simulink library "ammclib_bam_S32K3xx"  (R2016a)
settings: Solver=VariableStepAuto  SolverMode=SingleTasking  StartTime=0.0  StopTime=10.0  RelTol=1e-3
undefined symbols (not defined in the file or in its folder): a1, a2, ADCMaxError, autoCalcEn, b0, b1, b2, cfg, dgain, escale, f16A1, f16A2, f16ADCMaxError, f16B0, f16B1, f16B2, f16C1, f16CC1sc, f16CC1sc_D, f16CC1sc_Q, f16CC2sc, f16CC2sc_D, f16CC2sc_Q, f16DerivGain, f16EGain, f16FiltCoef, f16HystOff, f16HystOn, f16IGain, f16IntegGain, f16IntegGain_D, f16IntegGain_Q, f16IntegGainQ, f16Kd, f16KLs, f16Kq, f16KRs, f16Limit, f16LowerLimit, f16LowerLimit_D, f16LowerLimit_Q, f16LowerLimitQ, f16ModIndex, f16OutValOff, f16OutValOn, f16PropGain, f16PropGain_D, f16PropGain_Q, f16PropGainQ, f16RampDown, f16RampUp, f16UGain, f16UpperLimit, f16UpperLimit_D, f16UpperLimit_Q, f16UpperLimitQ, f16WIGain, f32A1, f32A2, f32ADCMaxError ... (+180)
(part 22 of 50)

== system ammclib_bam_S32K3xx/AMCLIB/FLT ==
  AMCLIB_BemfObsrvDQ_FLT : Subsystem  StartFcn=|  TreatAsAtomicUnit=on  mask(AMCLIB_BemfObsrvDQ_FLT){showStates=Hide (faster execution), resetStatesEnable=Pre-set according to the first set of inputs after reset, SampleTime=-1, intmethod=Trapezoidal, if0=350, iksi=1, Ld=3e-4, Lq=3e-4, Rs=0.33, mechspeed=3000, polepairs=1, autoCalcEn=on, fltIGain=0, fltUGain=0, fltWIGain=0, fltEGain=0, fltCC1sc_D=0, fltCC2sc_D=0, fltUpperLimit_D=0, fltLowerLimit_D=0, fltCC1sc_Q=0, fltCC2sc_Q=0, fltUpperLimit_Q=0, fltLowerLimit_Q=0, SampleTime_1=NaN}
      | ts=get_param(gcb,'CompiledSampleTime');
      | if iscell(ts)
      |   ts=ts{1};
      |   if iscell(ts)
      |     ts=ts{1};
      |   end
      | end
      | ts=ts(1);
      | set_param(gcb,'SampleTime_1',num2str(ts));
      | p=Simulink.Mask.get(gcb);
      | hintText=p.getDialogControl('timeHint');
      | SampleTime=Simulink.data.evalinGlobal(bdroot,get_param(gcb,'SampleTime'));
      | p=Simulink.Mask.get(gcb);
      | autoCalcEn=get_param(gcb,'autoCalcEn');
      | if strcmp(autoCalcEn,'on')
      |   if SampleTime==-1
      |     hintText.Prompt='Caution: Implementation parameters depend on inherited sample time. Make sure that the sample time of the block''s inputs corresponds to the sampling period in the target application.';
      |   else
      |     hintText.Prompt='Caution: Implementation parameters depend on the sample time. Make sure that the simulation time step corresponds to the sampling period in the target application.';
      |   end
      |   SampleTime=ts;
      |   fltIGain_bkup=get_param(gcb,'fltIGain');
      |   fltUGain_bkup=get_param(gcb,'fltUGain');
      |   fltWIGain_bkup=get_param(gcb,'fltWIGain');
      |   fltEGain_bkup=get_param(gcb,'fltEGain');
      |   fltCC1sc_D_bkup=get_param(gcb,'fltCC1sc_D');
      |   fltCC2sc_D_bkup=get_param(gcb,'fltCC2sc_D');
      |   fltUpperLimit_D_bkup=get_param(gcb,'fltUpperLimit_D');
      |   fltLowerLimit_D_bkup=get_param(gcb,'fltLowerLimit_D');
      |   fltCC1sc_Q_bkup=get_param(gcb,'fltCC1sc_Q');
      |   fltCC2sc_Q_bkup=get_param(gcb,'fltCC2sc_Q');
      |   fltUpperLimit_Q_bkup=get_param(gcb,'fltUpperLimit_Q');
      |   fltLowerLimit_Q_bkup=get_param(gcb,'fltLowerLimit_Q');
      |   intmethod=get_param(gcb,'intmethod');
      |   if0=Simulink.data.evalinGlobal(bdroot,get_param(gcb,'if0'));
      |   iksi=Simulink.data.evalinGlobal(bdroot,get_param(gcb,'iksi'));
      |   Ld=Simulink.data.evalinGlobal(bdroot,get_param(gcb,'Ld'));
      |   Lq=Simulink.data.evalinGlobal(bdroot,get_param(gcb,'Lq'));
      |   Rs=Simulink.data.evalinGlobal(bdroot,get_param(gcb,'Rs'));
      |   mechspeed=Simulink.data.evalinGlobal(bdroot,get_param(gcb,'mechspeed'));
      |   polepairs=Simulink.data.evalinGlobal(bdroot,get_param(gcb,'polepairs'));
      |   if (if0<=0)
      |     warning('Natural frequency f0 must be positive.');
      |   end
      |   if (iksi<=0)
      |     warning('Current loop attenuation must be positive.');
      |   end
      |   if (iksi>1)
      |     warning('Current loop attenuation must not exceed 1.');
      |   end
      |   if (Ld<=0)
      |     warning('Inductance Ld must be positive.');
      |   end
      |   if (Lq<=0)
      |     warning('Inductance Lq must be positive.');
      |   end
      |   if (Rs<0)
      |     warning('Resistance Rs must be non-negative.');
      |   end
      |   if (mechspeed<=0)
      |     warning('Max. speed must be positive.');
      |   end
      |   if (polepairs<1)
      |     warning('Number of pole pairs must be a natural number (1, 2, 3, ...).');
      |   end
      |   if (round(polepairs)~=polepairs)
      |     warning('Number of pole pairs must be a natural number (1, 2, 3, ...).');
      |   end
      |   w0=6.283185307179586*if0;
      |   pgain=2.0*iksi*w0*Ld-Rs;
      |   igain=w0*w0*Ld;
      |   if strcmp(intmethod,'Forward Rectangular')
      |     cc1=pgain;
      |     cc2=-pgain+igain*SampleTime;
      |   else
      |     if strcmp(intmethod,'Backward Rectangular')
      |       cc1=pgain+igain*SampleTime;
      |       cc2=-pgain;
      |     else
      |       cc1=pgain+igain*SampleTime*0.5;
      |       cc2=-pgain+igain*SampleTime*0.5;
      |     end
      |   end
      |   fltCC1sc_D=cc1;
      |   fltCC2sc_D=cc2;
      |   fltCC1sc_Q=fltCC1sc_D;
      |   fltCC2sc_Q=fltCC2sc_D;
      |   fltLowerLimit_D=-1000000.0;
      |   fltUpperLimit_D=1000000.0;
      |   fltLowerLimit_Q=fltLowerLimit_D;
      |   fltUpperLimit_Q=fltUpperLimit_D;
      |   fltIGain=(2.0*Ld-SampleTime*Rs)/(2.0*Ld+SampleTime*Rs);
      |   fltUGain=SampleTime/(2.0*Ld+SampleTime*Rs);
      |   fltWIGain=SampleTime*Lq/(2.0*Ld+SampleTime*Rs);
      |   fltEGain=SampleTime/(2.0*Ld+SampleTime*Rs);
      |   if isnan(fltIGain)
      |     if ~strcmp(fltIGain_bkup,'0')
      |       set_param(gcb,'fltIGain','0');
      |     end
      |   else
      |     tmps=num2str(fltIGain);
      |     if ~strcmp(fltIGain_bkup,tmps)
      |       set_param(gcb,'fltIGain',tmps);
      |     end
      |   end
      |   if isnan(fltUGain)
      |     if ~strcmp(fltUGain_bkup,'0')
      |       set_param(gcb,'fltUGain','0');
      |     end
      |   else
      |     tmps=num2str(fltUGain);
      |     if ~strcmp(fltUGain_bkup,tmps)
      |       set_param(gcb,'fltUGain',tmps);
      |     end
      |   end
      |   if isnan(fltWIGain)
      |     if ~strcmp(fltWIGain_bkup,'0')
      |       set_param(gcb,'fltWIGain','0');
      |     end
      |   else
      |     tmps=num2str(fltWIGain);
      |     if ~strcmp(fltWIGain_bkup,tmps)
      |       set_param(gcb,'fltWIGain',tmps);
      |     end
      |   end
      |   if isnan(fltEGain)
      |     if ~strcmp(fltEGain_bkup,'0')
      |       set_param(gcb,'fltEGain','0');
      |     end
      |   else
      |     tmps=num2str(fltEGain);
      |     if ~strcmp(fltEGain_bkup,tmps)
      |       set_param(gcb,'fltEGain',tmps);
      |     end
      |   end
      |   if isnan(fltCC1sc_D)
      |     if ~strcmp(fltCC1sc_D_bkup,'0')
      |       set_param(gcb,'fltCC1sc_D','0');
      |     end
      |   else
      |     tmps=num2str(fltCC1sc_D);
      |     if ~strcmp(fltCC1sc_D_bkup,tmps)
      |       set_param(gcb,'fltCC1sc_D',tmps);
      |     end
      |   end
      |   if isnan(fltCC2sc_D)
      |     if ~strcmp(fltCC2sc_D_bkup,'0')
      |       set_param(gcb,'fltCC2sc_D','0');
      |     end
      |   else
      |     tmps=num2str(fltCC2sc_D);
      |     if ~strcmp(fltCC2sc_D_bkup,tmps)
      |       set_param(gcb,'fltCC2sc_D',tmps);
      |     end
      |   end
      |   if isnan(fltUpperLimit_D)
      |     if ~strcmp(fltUpperLimit_D_bkup,'0')
      |       set_param(gcb,'fltUpperLimit_D','0');
      |     end
      |   else
      |     tmps=num2str(fltUpperLimit_D);
      |     if ~strcmp(fltUpperLimit_D_bkup,tmps)
      |       set_param(gcb,'fltUpperLimit_D',tmps);
      |     end
      |   end
      |   if isnan(fltLowerLimit_D)
      |     if ~strcmp(fltLowerLimit_D_bkup,'0')
      |       set_param(gcb,'fltLowerLimit_D','0');
      |     end
      |   else
      |     tmps=num2str(fltLowerLimit_D);
      |     if ~strcmp(fltLowerLimit_D_bkup,tmps)
      |       set_param(gcb,'fltLowerLimit_D',tmps);
      |     end
      |   end
      |   if isnan(fltCC1sc_Q)
      |     if ~strcmp(fltCC1sc_Q_bkup,'0')
      |       set_param(gcb,'fltCC1sc_Q','0');
      |     end
      |   else
      |     tmps=num2str(fltCC1sc_Q);
      |     if ~strcmp(fltCC1sc_Q_bkup,tmps)
      |       set_param(gcb,'fltCC1sc_Q',tmps);
      |     end
      |   end
      |   if isnan(fltCC2sc_Q)
      |     if ~strcmp(fltCC2sc_Q_bkup,'0')
      |       set_param(gcb,'fltCC2sc_Q','0');
      |     end
      |   else
      |     tmps=num2str(fltCC2sc_Q);
      |     if ~strcmp(fltCC2sc_Q_bkup,tmps)
      |       set_param(gcb,'fltCC2sc_Q',tmps);
      |     end
      |   end
      |   if isnan(fltUpperLimit_Q)
      |     if ~strcmp(fltUpperLimit_Q_bkup,'0')
      |       set_param(gcb,'fltUpperLimit_Q','0');
      |     end
      |   else
      |     tmps=num2str(fltUpperLimit_Q);
      |     if ~strcmp(fltUpperLimit_Q_bkup,tmps)
      |       set_param(gcb,'fltUpperLimit_Q',tmps);
      |     end
      |   end
      |   if isnan(fltLowerLimit_Q)
      |     if ~strcmp(fltLowerLimit_Q_bkup,'0')
      |       set_param(gcb,'fltLowerLimit_Q','0');
      |     end
      |   else
      |     tmps=num2str(fltLowerLimit_Q);
      |     if ~strcmp(fltLowerLimit_Q_bkup,tmps)
      |       set_param(gcb,'fltLowerLimit_Q',tmps);
      |     end
      |   end
      | end
      mask prompts: showStates "Show internal states:"; resetStatesEnable "Internal state after reset:"; SampleTime "Sample time (-1 for inherited):"; intmethod "Integration method:"; if0 "Current loop natural frequency f0 [Hz]:"; iksi "Current loop attenuation ξ:"; Ld "D-axis stator inductance Ld [H]"; Lq "Q-axis stator inductance Lq [H]"; Rs "Winding resistance Rs [ohm]:"; mechspeed "Maximum mechanical speed of the motor [RPM]:"; polepairs "Number of pole pairs of the motor:"; autoCalcEn "Calculate implementation parameters from physical parameters"; fltIGain "fltIGain (RL circuit constant):"; fltUGain "fltUGain (Voltage cross-coupling constant):"; fltWIGain "fltWIGain (Angular velocity cross-coupling constant):"; fltEGain "fltEGain (Back-EMF cross-coupling constant):"; fltCC1sc_D "fltCC1sc_D (CC1 coefficient of the D-axis PI controller):"; fltCC2sc_D "fltCC2sc_D (CC2 coefficient of the D-axis PI controller):"; fltUpperLimit_D "fltUpperLimit_D (Upper Limit of the D-axis PI controller):"; fltLowerLimit_D "fltLowerLimit_D (Lower Limit of the D-axis PI controller):"; fltCC1sc_Q "fltCC1sc_Q (CC1 coefficient of the Q-axis PI controller):"; fltCC2sc_Q "fltCC2sc_Q (CC2 coefficient of the Q-axis PI controller):"; fltUpperLimit_Q "fltUpperLimit_Q (Upper Limit of the Q-axis PI controller):"; fltLowerLimit_Q "fltLowerLimit_Q (Lower Limit of the Q-axis PI controller):"; SampleTime_1 "Discrete sample time:"
      mask help: PMSM back-EMF observer DQ in single precision floating-point implementation. This block supports re-initialization of the internal state during simulation. If the block is reset, the observer will align with the motor's position and speed measured in the next time step. This allows seamless on-the-fly transition to the closed-loop control. Refer to the AMMCLIB User's Guide for further details.
      mask init:
      | ddName = get_param(bdroot,'DataDictionary');
      | if length(ddName)==0
      |   set_param(bdroot,'DataDictionary','ammclib_types.sldd');
      | else
      |   dd = Simulink.data.dictionary.open(ddName);
      |   data = getSection(dd,'Design Data');
      |   if ~exist(data,'SWLIBS_2Syst_F16')
      |     addDataSource(dd,'ammclib_types.sldd');
      |     saveChanges(dd);
      |   end
      | end
      | 
      | if showStates == 1
      |   % hidden state variables
      |   if strcmp(get_param([gcb '/fltIGain'], 'BlockType'), 'Inport')
      |     posblk = get_param(gcb, 'Position');
      | 
      |     pos = get_param([gcb, '/fltIGain'], 'Position');
      |     orient = get_param([gcb, '/fltIGain'], 'Orientation');
      |     delete_block([gcb, '/fltIGain']);
      |     add_block('built-in/Ground', [gcb, '/fltIGain'], 'Position', pos, 'Orientation', orient);
      | 
      |     pos = get_param([gcb, '/fltUGain'], 'Position');
      |     orient = get_param([gcb, '/fltUGain'], 'Orientation');
      |     delete_block([gcb, '/fltUGain']);
      |     add_block('built-in/Ground', [gcb, '/fltUGain'], 'Position', pos, 'Orientation', orient);
      | 
      |     pos = get_param([gcb, '/fltWIGain'], 'Position');
      |     orient = get_param([gcb, '/fltWIGain'], 'Orientation');
      |     delete_block([gcb, '/fltWIGain']);
      |     add_block('built-in/Ground', [gcb, '/fltWIGain'], 'Position', pos, 'Orientation', orient);
      | 
      |     pos = get_param([gcb, '/fltEGain'], 'Position');
      |     orient = get_param([gcb, '/fltEGain'], 'Orientation');
      |     delete_block([gcb, '/fltEGain']);
      |     add_block('built-in/Ground', [gcb, '/fltEGain'], 'Position', pos, 'Orientation', orient);
      | 
      |     pos = get_param([gcb, '/fltCC1sc_D'], 'Position');
      |     orient = get_param([gcb, '/fltCC1sc_D'], 'Orientation');
      |     delete_block([gcb, '/fltCC1sc_D']);
      |     add_block('built-in/Ground', [gcb, '/fltCC1sc_D'], 'Position', pos, 'Orientation', orient);
      | 
      |     pos = get_param([gcb, '/fltCC2sc_D'], 'Position');
      |     orient = get_param([gcb, '/fltCC2sc_D'], 'Orientation');
      |     delete_block([gcb, '/fltCC2sc_D']);
      |     add_block('built-in/Ground', [gcb, '/fltCC2sc_D'], 'Position', pos, 'Orientation', orient);
      | 
      |     pos = get_param([gcb, '/fltUpperLimit_D'], 'Position');
      |     orient = get_param([gcb, '/fltUpperLimit_D'], 'Orientation');
      |     delete_block([gcb, '/fltUpperLimit_D']);
      |     add_block('built-in/Ground', [gcb, '/fltUpperLimit_D'], 'Position', pos, 'Orientation', orient);
      | 
      |     pos = get_param([gcb, '/fltLowerLimit_D'], 'Position');
      |     orient = get_param([gcb, '/fltLowerLimit_D'], 'Orientation');
      |     delete_block([gcb, '/fltLowerLimit_D']);
      |     add_block('built-in/Ground', [gcb, '/fltLowerLimit_D'], 'Position', pos, 'Orientation', orient);
      | 
      |     pos = get_param([gcb, '/fltCC1sc_Q'], 'Position');
      |     orient = get_param([gcb, '/fltCC1sc_Q'], 'Orientation');
      |     delete_block([gcb, '/fltCC1sc_Q']);
      |     add_block('built-in/Ground', [gcb, '/fltCC1sc_Q'], 'Position', pos, 'Orientation', orient);
      | 
      |     pos = get_param([gcb, '/fltCC2sc_Q'], 'Position');
      |     orient = get_param([gcb, '/fltCC2sc_Q'], 'Orientation');
      |     delete_block([gcb, '/fltCC2sc_Q']);
      |     add_block('built-in/Ground', [gcb, '/fltCC2sc_Q'], 'Position', pos, 'Orientation', orient);
      | 
      |     pos = get_param([gcb, '/fltUpperLimit_Q'], 'Position');
      |     orient = get_param([gcb, '/fltUpperLimit_Q'], 'Orientation');
      |     delete_block([gcb, '/fltUpperLimit_Q']);
      |     add_block('built-in/Ground', [gcb, '/fltUpperLimit_Q'], 'Position', pos, 'Orientation', orient);
      | 
      |     pos = get_param([gcb, '/fltLowerLimit_Q'], 'Position');
      |     orient = get_param([gcb, '/fltLowerLimit_Q'], 'Orientation');
      |     delete_block([gcb, '/fltLowerLimit_Q']);
      |     add_block('built-in/Ground', [gcb, '/fltLowerLimit_Q'], 'Position', pos, 'Orientation', orient);
      | 
      |     pos = get_param([gcb, '/fltAcc_D'], 'Position');
      |     orient = get_param([gcb, '/fltAcc_D'], 'Orientation');
      |     delete_block([gcb, '/fltAcc_D']);
      |     add_block('built-in/Ground', [gcb, '/fltAcc_D'], 'Position', pos, 'Orientation', orient);
      | 
      |     pos = get_param([gcb, '/fltInErrK1_D'], 'Position');
      |     orient = get_param([gcb, '/fltInErrK1_D'], 'Orientation');
      |     delete_block([gcb, '/fltInErrK1_D']);
      |     add_block('built-in/Ground', [gcb, '/fltInErrK1_D'], 'Position', pos, 'Orientation', orient);
      | 
      |     pos = get_param([gcb, '/fltAcc_Q'], 'Position');
      |     orient = get_param([gcb, '/fltAcc_Q'], 'Orientation');
      |     delete_block([gcb, '/fltAcc_Q']);
      |     add_block('built-in/Ground', [gcb, '/fltAcc_Q'], 'Position', pos, 'Orientation', orient);
      | 
      |     pos = get_param([gcb, '/fltInErrK1_Q'], 'Position');
      |     orient = get_param([gcb, '/fltInErrK1_Q'], 'Orientation');
      |     delete_block([gcb, '/fltInErrK1_Q']);
      |     add_block('built-in/Ground', [gcb, '/fltInErrK1_Q'], 'Position', pos, 'Orientation', orient);
      | 
      |     pos = get_param([gcb, '/fltIObsrvIn_1_D'], 'Position');
      |     orient = get_param([gcb, '/fltIObsrvIn_1_D'], 'Orientation');
      |     delete_block([gcb, '/fltIObsrvIn_1_D']);
      |     add_block('built-in/Ground', [gcb, '/fltIObsrvIn_1_D'], 'Position', pos, 'Orientation', orient);
      | 
      |     pos = get_param([gcb, '/fltIObsrvIn_1_Q'], 'Position');
      |     orient = get_param([gcb, '/fltIObsrvIn_1_Q'], 'Orientation');
      |     delete_block([gcb, '/fltIObsrvIn_1_Q']);
      |     add_block('built-in/Ground', [gcb, '/fltIObsrvIn_1_Q'], 'Position', pos, 'Orientation', orient);
      | 
      |     pos = get_param([gcb, '/fltIObsrv_D'], 'Position');
      |     orient = get_param([gcb, '/fltIObsrv_D'], 'Orientation');
      |     delete_block([gcb, '/fltIObsrv_D']);
      |     add_block('built-in/Ground', [gcb, '/fltIObsrv_D'], 'Position', pos, 'Orientation', orient);
      | 
      |     pos = get_param([gcb, '/fltIObsrv_Q'], 'Position');
      |     orient = get_param([gcb, '/fltIObsrv_Q'], 'Orientation');
      |     delete_block([gcb, '/fltIObsrv_Q']);
      |     add_block('built-in/Ground', [gcb, '/fltIObsrv_Q'], 'Position', pos, 'Orientation', orient);
      | 
      | 
      |     pmask=Simulink.Mask.get(gcb);
      |     pctrl=pmask.getParameter('SampleTime');
      |     pctrl.set('TypeOptions',{'pIAB/SampleTime','pUAB/SampleTime','fltVelocity/SampleTime','fltPhase/SampleTime'});
      | 
      |     pos = get_param([gcb '/fltEObsrv_D_Out'], 'Position');
      |     orient = get_param([gcb '/fltEObsrv_D_Out'], 'Orientation');
      |     delete_block([gcb '/fltEObsrv_D_Out']);
      |     add_block('built-in/Terminator', [gcb '/fltEObsrv_D_Out'], 'Position', pos, 'Orientation', orient);
      | 
      |     pos = get_param([gcb '/fltEObsrv_Q_Out'], 'Position');
      |     orient = get_param([gcb '/fltEObsrv_Q_Out'], 'Orientation');
      |     delete_block([gcb '/fltEObsrv_Q_Out']);
      |     add_block('built-in/Terminator', [gcb '/fltEObsrv_Q_Out'], 'Position', pos, 'Orientation', orient);
      | 
      |     pos = get_param([gcb '/fltAcc_D_Out'], 'Position');
      |     orient = get_param([gcb '/fltAcc_D_Out'], 'Orientation');
      |     delete_block([gcb '/fltAcc_D_Out']);
      |     add_block('built-in/Terminator', [gcb '/fltAcc_D_Out'], 'Position', pos, 'Orientation', orient);
      | 
      |     pos = get_param([gcb '/fltInErrK1_D_Out'], 'Position');
      |     orient = get_param([gcb '/fltInErrK1_D_Out'], 'Orientation');
      |     delete_block([gcb '/fltInErrK1_D_Out']);
      |     add_block('built-in/Terminator', [gcb '/fltInErrK1_D_Out'], 'Position', pos, 'Orientation', orient);
      | 
      |     pos = get_param([gcb '/fltAcc_Q_Out'], 'Position');
      |     orient = get_param([gcb '/fltAcc_Q_Out'], 'Orientation');
      |     delete_block([gcb '/fltAcc_Q_Out']);
      |     add_block('built-in/Terminator', [gcb '/fltAcc_Q_Out'], 'Position', pos, 'Orientation', orient);
      | 
      |     pos = get_param([gcb '/fltInErrK1_Q_Out'], 'Position');
      |     orient = get_param([gcb '/fltInErrK1_Q_Out'], 'Orientation');
      |     delete_block([gcb '/fltInErrK1_Q_Out']);
      |     add_block('built-in/Terminator', [gcb '/fltInErrK1_Q_Out'], 'Position', pos, 'Orientation', orient);
      | 
      |     pos = get_param([gcb '/fltIObsrvIn_1_D_Out'], 'Position');
      |     orient = get_param([gcb '/fltIObsrvIn_1_D_Out'], 'Orientation');
      |     delete_block([gcb '/fltIObsrvIn_1_D_Out']);
      |     add_block('built-in/Terminator', [gcb '/fltIObsrvIn_1_D_Out'], 'Position', pos, 'Orientation', orient);
      | 
      |     pos = get_param([gcb '/fltIObsrvIn_1_Q_Out'], 'Position');
      |     orient = get_param([gcb '/fltIObsrvIn_1_Q_Out'], 'Orientation');
      |     delete_block([gcb '/fltIObsrvIn_1_Q_Out']);
      |     add_block('built-in/Terminator', [gcb '/fltIObsrvIn_1_Q_Out'], 'Position', pos, 'Orientation', orient);
      | 
      |     pos = get_param([gcb '/fltIObsrv_D_Out'], 'Position');
      |     orient = get_param([gcb '/fltIObsrv_D_Out'], 'Orientation');
      |     delete_block([gcb '/fltIObsrv_D_Out']);
      |     add_block('built-in/Terminator', [gcb '/fltIObsrv_D_Out'], 'Position', pos, 'Orientation', orient);
      | 
      |     pos = get_param([gcb '/fltIObsrv_Q_Out'], 'Position');
      |     orient = get_param([gcb '/fltIObsrv_Q_Out'], 'Orientation');
      |     delete_block([gcb '/fltIObsrv_Q_Out']);
      |     add_block('built-in/Terminator', [gcb '/fltIObsrv_Q_Out'], 'Position', pos, 'Orientation', orient);
      | 
      |     set_param([gcb '/pIAB'], 'Port', '1');
      |     set_param([gcb '/pUAB'], 'Port', '2');
      |     set_param([gcb '/fltVelocity'], 'Port', '3');
      |     set_param([gcb '/fltPhase'], 'Port', '4');
      | 
      |     tmpOutCnt=0;
      |     tmpOutCnt=tmpOutCnt+1;
      |     set_param([gcb '/fltPhaseErr'], 'Port', num2str(tmpOutCnt));
      | 
      |     autoCalcEn=get_param(gcb,'autoCalcEn');
      |     if strcmp(autoCalcEn,'on')
      |       set_param(gcb,'MaskEnables',{'on','on','on','on','on','on','on','on','on','on','on','on','on','on','on','on','on','on','on','on','on','on','on','on','off'});
      |     else
      |       set_param(gcb,'MaskEnables',{'on','on','on','off','off','off','off','off','off','off','off','on','on','on','on','on','on','on','on','on','on','on','on','on','off'});
      |     end
      | 
      |     if (posblk(4) - posblk(2)) > 125
      |       height = 125;
      |       set_param(gcb,'Position',[posblk(1), posblk(2), posblk(3), posblk(2)+height])
      |     end
      |   end
      | else
      |   % shown state variables
      |   if strcmp(get_param([gcb '/fltIGain'], 'BlockType'), 'Ground')
      |     posblk = get_param(gcb, 'Position');
      | 
      |     pos = get_param([gcb, '/fltIGain'], 'Position');
      |     orient = get_param([gcb, '/fltIGain'], 'Orientation');
      |     delete_block([gcb, '/fltIGain']);
      |     add_block('built-in/Inport', [gcb, '/fltIGain'], 'Position', pos, 'Orientation', orient, 'OutDataTypeStr', 'single');
      | 
      |     pos = get_param([gcb, '/fltUGain'], 'Position');
      |     orient = get_param([gcb, '/fltUGain'], 'Orientation');
      |     delete_block([gcb, '/fltUGain']);
      |     add_block('built-in/Inport', [gcb, '/fltUGain'], 'Position', pos, 'Orientation', orient, 'OutDataTypeStr', 'single');
      | 
      |     pos = get_param([gcb, '/fltWIGain'], 'Position');
      |     orient = get_param([gcb, '/fltWIGain'], 'Orientation');
      |     delete_block([gcb, '/fltWIGain']);
      |     add_block('built-in/Inport', [gcb, '/fltWIGain'], 'Position', pos, 'Orientation', orient, 'OutDataTypeStr', 'single');
      | 
      |     pos = get_param([gcb, '/fltEGain'], 'Position');
      |     orient = get_param([gcb, '/fltEGain'], 'Orientation');
      |     delete_block([gcb, '/fltEGain']);
      |     add_block('built-in/Inport', [gcb, '/fltEGain'], 'Position', pos, 'Orientation', orient, 'OutDataTypeStr', 'single');
      | 
      |     pos = get_param([gcb, '/fltCC1sc_D'], 'Position');
      |     orient = get_param([gcb, '/fltCC1sc_D'], 'Orientation');
      |     delete_block([gcb, '/fltCC1sc_D']);
      |     add_block('built-in/Inport', [gcb, '/fltCC1sc_D'], 'Position', pos, 'Orientation', orient, 'OutDataTypeStr', 'single');
      | 
      |     pos = get_param([gcb, '/fltCC2sc_D'], 'Position');
      |     orient = get_param([gcb, '/fltCC2sc_D'], 'Orientation');
      |     delete_block([gcb, '/fltCC2sc_D']);
      |     add_block('built-in/Inport', [gcb, '/fltCC2sc_D'], 'Position', pos, 'Orientation', orient, 'OutDataTypeStr', 'single');
      | 
      |     pos = get_param([gcb, '/fltUpperLimit_D'], 'Position');
      |     orient = get_param([gcb, '/fltUpperLimit_D'], 'Orientation');
      |     delete_block([gcb, '/fltUpperLimit_D']);
      |     add_block('built-in/Inport', [gcb, '/fltUpperLimit_D'], 'Position', pos, 'Orientation', orient, 'OutDataTypeStr', 'single');
      | 
      |     pos = get_param([gcb, '/fltLowerLimit_D'], 'Position');
      |     orient = get_param([gcb, '/fltLowerLimit_D'], 'Orientation');
      |     delete_block([gcb, '/fltLowerLimit_D']);
      |     add_block('built-in/Inport', [gcb, '/fltLowerLimit_D'], 'Position', pos, 'Orientation', orient, 'OutDataTypeStr', 'single');
      | 
      |     pos = get_param([gcb, '/fltCC1sc_Q'], 'Position');
      |     orient = get_param([gcb, '/fltCC1sc_Q'], 'Orientation');
      |     delete_block([gcb, '/fltCC1sc_Q']);
      |     add_block('built-in/Inport', [gcb, '/fltCC1sc_Q'], 'Position', pos, 'Orientation', orient, 'OutDataTypeStr', 'single');
      | 
      |     pos = get_param([gcb, '/fltCC2sc_Q'], 'Position');
      |     orient = get_param([gcb, '/fltCC2sc_Q'], 'Orientation');
      |     delete_block([gcb, '/fltCC2sc_Q']);
      |     add_block('built-in/Inport', [gcb, '/fltCC2sc_Q'], 'Position', pos, 'Orientation', orient, 'OutDataTypeStr', 'single');
      | 
      |     pos = get_param([gcb, '/fltUpperLimit_Q'], 'Position');
      |     orient = get_param([gcb, '/fltUpperLimit_Q'], 'Orientation');
      |     delete_block([gcb, '/fltUpperLimit_Q']);
      |     add_block('built-in/Inport', [gcb, '/fltUpperLimit_Q'], 'Position', pos, 'Orientation', orient, 'OutDataTypeStr', 'single');
      | 
      |     pos = get_param([gcb, '/fltLowerLimit_Q'], 'Position');
      |     orient = get_param([gcb, '/fltLowerLimit_Q'], 'Orientation');
      |     delete_block([gcb, '/fltLowerLimit_Q']);
      |     add_block('built-in/Inport', [gcb, '/fltLowerLimit_Q'], 'Position', pos, 'Orientation', orient, 'OutDataTypeStr', 'single');
      | 
      |     pos = get_param([gcb, '/fltAcc_D'], 'Position');
      |     orient = get_param([gcb, '/fltAcc_D'], 'Orientation');
      |     delete_block([gcb, '/fltAcc_D']);
      |     add_block('built-in/Inport', [gcb, '/fltAcc_D'], 'Position', pos, 'Orientation', orient, 'OutDataTypeStr', 'single');
      | 
      |     pos = get_param([gcb, '/fltInErrK1_D'], 'Position');
      |     orient = get_param([gcb, '/fltInErrK1_D'], 'Orientation');
      |     delete_block([gcb, '/fltInErrK1_D']);
      |     add_block('built-in/Inport', [gcb, '/fltInErrK1_D'], 'Position', pos, 'Orientation', orient, 'OutDataTypeStr', 'single');
      | 
      |     pos = get_param([gcb, '/fltAcc_Q'], 'Position');
      |     orient = get_param([gcb, '/fltAcc_Q'], 'Orientation');
      |     delete_block([gcb, '/fltAcc_Q']);
      |     add_block('built-in/Inport', [gcb, '/fltAcc_Q'], 'Position', pos, 'Orientation', orient, 'OutDataTypeStr', 'single');
      | 
      |     pos = get_param([gcb, '/fltInErrK1_Q'], 'Position');
      |     orient = get_param([gcb, '/fltInErrK1_Q'], 'Orientation');
      |     delete_block([gcb, '/fltInErrK1_Q']);
      |     add_block('built-in/Inport', [gcb, '/fltInErrK1_Q'], 'Position', pos, 'Orientation', orient, 'OutDataTypeStr', 'single');
      | 
      |     pos = get_param([gcb, '/fltIObsrvIn_1_D'], 'Position');
      |     orient = get_param([gcb, '/fltIObsrvIn_1_D'], 'Orientation');
      |     delete_block([gcb, '/fltIObsrvIn_1_D']);
      |     add_block('built-in/Inport', [gcb, '/fltIObsrvIn_1_D'], 'Position', pos, 'Orientation', orient, 'OutDataTypeStr', 'single');
      | 
      |     pos = get_param([gcb, '/fltIObsrvIn_1_Q'], 'Position');
      |     orient = get_param([gcb, '/fltIObsrvIn_1_Q'], 'Orientation');
      |     delete_block([gcb, '/fltIObsrvIn_1_Q']);
      |     add_block('built-in/Inport', [gcb, '/fltIObsrvIn_1_Q'], 'Position', pos, 'Orientation', orient, 'OutDataTypeStr', 'single');
      | 
      |     pos = get_param([gcb, '/fltIObsrv_D'], 'Position');
      |     orient = get_param([gcb, '/fltIObsrv_D'], 'Orientation');
      |     delete_block([gcb, '/fltIObsrv_D']);
      |     add_block('built-in/Inport', [gcb, '/fltIObsrv_D'], 'Position', pos, 'Orientation', orient, 'OutDataTypeStr', 'single');
      | 
      |     pos = get_param([gcb, '/fltIObsrv_Q'], 'Position');
      |     orient = get_param([gcb, '/fltIObsrv_Q'], 'Orientation');
      |     delete_block([gcb, '/fltIObsrv_Q']);
      |     add_block('built-in/Inport', [gcb, '/fltIObsrv_Q'], 'Position', pos, 'Orientation', orient, 'OutDataTypeStr', 'single');
      | 
      | 
      | 
      |     pos = get_param([gcb '/fltEObsrv_D_Out'], 'Position');
      |     orient = get_param([gcb '/fltEObsrv_D_Out'], 'Orientation');
      |     delete_block([gcb '/fltEObsrv_D_Out']);
      |     add_block('built-in/Outport', [gcb '/fltEObsrv_D_Out'], 'Position', pos, 'Orientation', orient);
      | 
      |     pos = get_param([gcb '/fltEObsrv_Q_Out'], 'Position');
      |     orient = get_param([gcb '/fltEObsrv_Q_Out'], 'Orientation');
      |     delete_block([gcb '/fltEObsrv_Q_Out']);
      |     add_block('built-in/Outport', [gcb '/fltEObsrv_Q_Out'], 'Position', pos, 'Orientation', orient);
      | 
      |     pos = get_param([gcb '/fltAcc_D_Out'], 'Position');
      |     orient = get_param([gcb '/fltAcc_D_Out'], 'Orientation');
      |     delete_block([gcb '/fltAcc_D_Out']);
      |     add_block('built-in/Outport', [gcb '/fltAcc_D_Out'], 'Position', pos, 'Orientation', orient);
      | 
      |     pos = get_param([gcb '/fltInErrK1_D_Out'], 'Position');
      |     orient = get_param([gcb '/fltInErrK1_D_Out'], 'Orientation');
      |     delete_block([gcb '/fltInErrK1_D_Out']);
      |     add_block('built-in/Outport', [gcb '/fltInErrK1_D_Out'], 'Position', pos, 'Orientation', orient);
      | 
      |     pos = get_param([gcb '/fltAcc_Q_Out'], 'Position');
      |     orient = get_param([gcb '/fltAcc_Q_Out'], 'Orientation');
      |     delete_block([gcb '/fltAcc_Q_Out']);
      |     add_block('built-in/Outport', [gcb '/fltAcc_Q_Out'], 'Position', pos, 'Orientation', orient);
      | 
      |     pos = get_param([gcb '/fltInErrK1_Q_Out'], 'Position');
      |     orient = get_param([gcb '/fltInErrK1_Q_Out'], 'Orientation');
      |     delete_block([gcb '/fltInErrK1_Q_Out']);
      |     add_block('built-in/Outport', [gcb '/fltInErrK1_Q_Out'], 'Position', pos, 'Orientation', orient);
      | 
      |     pos = get_param([gcb '/fltIObsrvIn_1_D_Out'], 'Position');
      |     orient = get_param([gcb '/fltIObsrvIn_1_D_Out'], 'Orientation');
      |     delete_block([gcb '/fltIObsrvIn_1_D_Out']);
      |     add_block('built-in/Outport', [gcb '/fltIObsrvIn_1_D_Out'], 'Position', pos, 'Orientation', orient);
      | 
      |     pos = get_param([gcb '/fltIObsrvIn_1_Q_Out'], 'Position');
      |     orient = get_param([gcb '/fltIObsrvIn_1_Q_Out'], 'Orientation');
      |     delete_block([gcb '/fltIObsrvIn_1_Q_Out']);
      |     add_block('built-in/Outport', [gcb '/fltIObsrvIn_1_Q_Out'], 'Position', pos, 'Orientation', orient);
      | 
      |     pos = get_param([gcb '/fltIObsrv_D_Out'], 'Position');
      |     orient = get_param([gcb '/fltIObsrv_D_Out'], 'Orientation');
      |     delete_block([gcb '/fltIObsrv_D_Out']);
      |     add_block('built-in/Outport', [gcb '/fltIObsrv_D_Out'], 'Position', pos, 'Orientation', orient);
      | 
      |     pos = get_param([gcb '/fltIObsrv_Q_Out'], 'Position');
      |     orient = get_param([gcb '/fltIObsrv_Q_Out'], 'Orientation');
      |     delete_block([gcb '/fltIObsrv_Q_Out']);
      |     add_block('built-in/Outport', [gcb '/fltIObsrv_Q_Out'], 'Position', pos, 'Orientation', orient);
      | 
      | 
      |     pmask=Simulink.Mask.get(gcb);
      |     pctrl=pmask.getParameter('SampleTime');
      |     pctrl.set('TypeOptions',{'pIAB/SampleTime','pUAB/SampleTime','fltVelocity/SampleTime','fltPhase/SampleTime','fltIGain/SampleTime','fltUGain/SampleTime','fltWIGain/SampleTime','fltEGain/SampleTime','fltCC1sc_D/SampleTime','fltCC2sc_D/SampleTime','fltUpperLimit_D/SampleTime','fltLowerLimit_D/SampleTime','fltCC1sc_Q/SampleTime','fltCC2sc_Q/SampleTime','fltUpperLimit_Q/SampleTime','fltLowerLimit_Q/SampleTime','fltAcc_D/SampleTime','fltInErrK1_D/SampleTime','fltAcc_Q/SampleTime','fltInErrK1_Q/SampleTime','fltIObsrvIn_1_D/SampleTime','fltIObsrvIn_1_Q/SampleTime','fltIObsrv_D/SampleTime','fltIObsrv_Q/SampleTime'});
      | 
      |     set_param([gcb '/pIAB'], 'Port', '1');
      |     set_param([gcb '/pUAB'], 'Port', '2');
      |     set_param([gcb '/fltVelocity'], 'Port', '3');
      |     set_param([gcb '/fltPhase'], 'Port', '4');
      |     set_param([gcb '/fltIGain'], 'Port', '5');
      |     set_param([gcb '/fltUGain'], 'Port', '6');
      |     set_param([gcb '/fltWIGain'], 'Port', '7');
      |     set_param([gcb '/fltEGain'], 'Port', '8');
      |     set_param([gcb '/fltCC1sc_D'], 'Port', '9');
      |     set_param([gcb '/fltCC2sc_D'], 'Port', '10');
      |     set_param([gcb '/fltUpperLimit_D'], 'Port', '11');
      |     set_param([gcb '/fltLowerLimit_D'], 'Port', '12');
      |     set_param([gcb '/fltCC1sc_Q'], 'Port', '13');
      |     set_param([gcb '/fltCC2sc_Q'], 'Port', '14');
      |     set_param([gcb '/fltUpperLimit_Q'], 'Port', '15');
      |     set_param([gcb '/fltLowerLimit_Q'], 'Port', '16');
      |     set_param([gcb '/fltAcc_D'], 'Port', '17');
      |     set_param([gcb '/fltInErrK1_D'], 'Port', '18');
      |     set_param([gcb '/fltAcc_Q'], 'Port', '19');
      |     set_param([gcb '/fltInErrK1_Q'], 'Port', '20');
      |     set_param([gcb '/fltIObsrvIn_1_D'], 'Port', '21');
      |     set_param([gcb '/fltIObsrvIn_1_Q'], 'Port', '22');
      |     set_param([gcb '/fltIObsrv_D'], 'Port', '23');
      |     set_param([gcb '/fltIObsrv_Q'], 'Port', '24');
      | 
      |     tmpOutCnt=0;
      |     tmpOutCnt=tmpOutCnt+1;
      |     set_param([gcb '/fltPhaseErr'], 'Port', num2str(tmpOutCnt));
      |     tmpOutCnt=tmpOutCnt+1;
      |     set_param([gcb '/fltEObsrv_D_Out'], 'Port', num2str(tmpOutCnt));
      |     tmpOutCnt=tmpOutCnt+1;
      |     set_param([gcb '/fltEObsrv_Q_Out'], 'Port', num2str(tmpOutCnt));
      |     tmpOutCnt=tmpOutCnt+1;
      |     set_param([gcb '/fltAcc_D_Out'], 'Port', num2str(tmpOutCnt));
      |     tmpOutCnt=tmpOutCnt+1;
      |     set_param([gcb '/fltInErrK1_D_Out'], 'Port', num2str(tmpOutCnt));
      |     tmpOutCnt=tmpOutCnt+1;
      |     set_param([gcb '/fltAcc_Q_Out'], 'Port', num2str(tmpOutCnt));
      |     tmpOutCnt=tmpOutCnt+1;
      |     set_param([gcb '/fltInErrK1_Q_Out'], 'Port', num2str(tmpOutCnt));
      |     tmpOutCnt=tmpOutCnt+1;
      |     set_param([gcb '/fltIObsrvIn_1_D_Out'], 'Port', num2str(tmpOutCnt));
      |     tmpOutCnt=tmpOutCnt+1;
      |     set_param([gcb '/fltIObsrvIn_1_Q_Out'], 'Port', num2str(tmpOutCnt));
      |     tmpOutCnt=tmpOutCnt+1;
      |     set_param([gcb '/fltIObsrv_D_Out'], 'Port', num2str(tmpOutCnt));
      |     tmpOutCnt=tmpOutCnt+1;
      |     set_param([gcb '/fltIObsrv_Q_Out'], 'Port', num2str(tmpOutCnt));
      | 
      |     set_param(gcb,'MaskEnables',{'on','on','on','off','off','off','off','off','off','off','off','off','off','off','off','off','off','off','off','off','off','off','off','off','off'});
      | 
      |     if (posblk(4) - posblk(2)) < 625
      |       height = 625;
      |       set_param(gcb,'Position',[posblk(1), posblk(2), posblk(3), posblk(2)+height])
      |     end
      |   end
      | end
      settings: RTWSystemCode=Inline
      mask Help: web([fileparts(which('ammclib_bam_S32K3xx.slx')) '/../doc/S32K3XXMCLUG.pdf'], '-browser')
      mask TypeOptions showStates: Hide (faster execution) | Show (allows debugging; connect feedback loops manually)
      mask Callback showStates:
      | maskStr=get_param(gcb,'showStates');
      | if strcmp(maskStr,'Hide (faster execution)')
      |   if strcmp(get_param([gcb '/fltIGain'], 'BlockType'), 'Inport')
      |     autoCalcEn=get_param(gcb,'autoCalcEn');
      |     if strcmp(autoCalcEn,'on')
      |       set_param(gcb,'MaskEnables',{'on','on','on','on','on','on','on','on','on','on','on','on','on','on','on','on','on','on','on','on','on','on','on','on','off'});
      |     else
      |       set_param(gcb,'MaskEnables',{'on','on','on','off','off','off','off','off','off','off','off','on','on','on','on','on','on','on','on','on','on','on','on','on','off'});
      |     end
      |   end
      | else
      |   if strcmp(get_param([gcb '/fltIGain'], 'BlockType'), 'Ground')
      |     set_param(gcb,'MaskEnables',{'on','on','on','off','off','off','off','off','off','off','off','off','off','off','off','off','off','off','off','off','off','off','off','off','off'});
      |   end
      | end
      mask TypeOptions resetStatesEnable: Pre-set according to the first set of inputs after reset | Clear to zero
      mask TypeOptions SampleTime: pIAB/SampleTime | pUAB/SampleTime | fltVelocity/SampleTime | fltPhase/SampleTime
      mask Callback SampleTime:
      | p=Simulink.Mask.get(gcb);
      | hintText=p.getDialogControl('timeHint');
      | SampleTime=Simulink.data.evalinGlobal(bdroot,get_param(gcb,'SampleTime'));
      | SampleTime_1=str2double(get_param(gcb,'SampleTime_1'));
      | if (((SampleTime==-1) && (~contains(hintText.Prompt,'inherited'))) || ...
      |     ((SampleTime~=-1) && contains(hintText.Prompt,'inherited')) || ...
      |     ((SampleTime~=-1) && (SampleTime_1~=SampleTime)) || ...
      |     ((SampleTime_1~=-1) && contains(hintText.Prompt,'yet')))
      |   if ((SampleTime==-1) && (~contains(hintText.Prompt,'inherited')))
      |     set_param(gcb,'SampleTime_1',num2str(NaN));
      |     SampleTime_1=NaN;
      |   end
      |   if (SampleTime~=-1)
      |     set_param(gcb,'SampleTime_1',num2str(SampleTime));
      |     SampleTime_1=SampleTime;
      |   end
      |   autoCalcEn=get_param(gcb,'autoCalcEn');
      |   if strcmp(autoCalcEn,'on')
      |     p=Simulink.Mask.get(gcb);
      |     hintText=p.getDialogControl('timeHint');
      |     if SampleTime==-1
      |       SampleTime=SampleTime_1;
      |       if isnan(SampleTime)
      |         hintText.Prompt='Note: Implementation parameters cannot be calculated yet because the block''s inherited sample time is unknown. Simulink will update the sample time when you run the simulation.';
      |       else
      |         hintText.Prompt='Caution: Implementation parameters depend on inherited sample time. Make sure that the sample time of the block''s inputs corresponds to the sampling period in the target application.';
      |       end
      |     else
      |       hintText.Prompt='Caution: Implementation parameters depend on the sample time. Make sure that the simulation time step corresponds to the sampling period in the target application.';
      |     end
      |     fltIGain_bkup=get_param(gcb,'fltIGain');
      |     fltUGain_bkup=get_param(gcb,'fltUGain');
      |     fltWIGain_bkup=get_param(gcb,'fltWIGain');
      |     fltEGain_bkup=get_param(gcb,'fltEGain');
      |     fltCC1sc_D_bkup=get_param(gcb,'fltCC1sc_D');
      |     fltCC2sc_D_bkup=get_param(gcb,'fltCC2sc_D');
      |     fltUpperLimit_D_bkup=get_param(gcb,'fltUpperLimit_D');
      |     fltLowerLimit_D_bkup=get_param(gcb,'fltLowerLimit_D');
      |     fltCC1sc_Q_bkup=get_param(gcb,'fltCC1sc_Q');
      |     fltCC2sc_Q_bkup=get_param(gcb,'fltCC2sc_Q');
      |     fltUpperLimit_Q_bkup=get_param(gcb,'fltUpperLimit_Q');
      |     fltLowerLimit_Q_bkup=get_param(gcb,'fltLowerLimit_Q');
      |     intmethod=get_param(gcb,'intmethod');
      |     if0=Simulink.data.evalinGlobal(bdroot,get_param(gcb,'if0'));
      |     iksi=Simulink.data.evalinGlobal(bdroot,get_param(gcb,'iksi'));
      |     Ld=Simulink.data.evalinGlobal(bdroot,get_param(gcb,'Ld'));
      |     Lq=Simulink.data.evalinGlobal(bdroot,get_param(gcb,'Lq'));
      |     Rs=Simulink.data.evalinGlobal(bdroot,get_param(gcb,'Rs'));
      |     mechspeed=Simulink.data.evalinGlobal(bdroot,get_param(gcb,'mechspeed'));
      |     polepairs=Simulink.data.evalinGlobal(bdroot,get_param(gcb,'polepairs'));
      |     if (if0<=0)
      |       warning('Natural frequency f0 must be positive.');
      |     end
      |     if (iksi<=0)
      |       warning('Current loop attenuation must be positive.');
      |     end
      |     if (iksi>1)
      |       warning('Current loop attenuation must not exceed 1.');
      |     end
      |     if (Ld<=0)
      |       warning('Inductance Ld must be positive.');
      |     end
      |     if (Lq<=0)
      |       warning('Inductance Lq must be positive.');
      |     end
      |     if (Rs<0)
      |       warning('Resistance Rs must be non-negative.');
      |     end
      |     if (mechspeed<=0)
      |       warning('Max. speed must be positive.');
      |     end
      |     if (polepairs<1)
      |       warning('Number of pole pairs must be a natural number (1, 2, 3, ...).');
      |     end
      |     if (round(polepairs)~=polepairs)
      |       warning('Number of pole pairs must be a natural number (1, 2, 3, ...).');
      |     end
      |     w0=6.283185307179586*if0;
      |     pgain=2.0*iksi*w0*Ld-Rs;
      |     igain=w0*w0*Ld;
      |     if strcmp(intmethod,'Forward Rectangular')
      |       cc1=pgain;
      |       cc2=-pgain+igain*SampleTime;
      |     else
      |       if strcmp(intmethod,'Backward Rectangular')
      |         cc1=pgain+igain*SampleTime;
      |         cc2=-pgain;
      |       else
      |         cc1=pgain+igain*SampleTime*0.5;
      |         cc2=-pgain+igain*SampleTime*0.5;
      |       end
      |     end
      |     fltCC1sc_D=cc1;
      |     fltCC2sc_D=cc2;
      |     fltCC1sc_Q=fltCC1sc_D;
      |     fltCC2sc_Q=fltCC2sc_D;
      |     fltLowerLimit_D=-1000000.0;
      |     fltUpperLimit_D=1000000.0;
      |     fltLowerLimit_Q=fltLowerLimit_D;
      |     fltUpperLimit_Q=fltUpperLimit_D;
      |     fltIGain=(2.0*Ld-SampleTime*Rs)/(2.0*Ld+SampleTime*Rs);
      |     fltUGain=SampleTime/(2.0*Ld+SampleTime*Rs);
      |     fltWIGain=SampleTime*Lq/(2.0*Ld+SampleTime*Rs);
      |     fltEGain=SampleTime/(2.0*Ld+SampleTime*Rs);
      |     if isnan(fltIGain)
      |       if ~strcmp(fltIGain_bkup,'0')
      |         set_param(gcb,'fltIGain','0');
      |       end
      |     else
      |       tmps=num2str(fltIGain);
      |       if ~strcmp(fltIGain_bkup,tmps)
      |         set_param(gcb,'fltIGain',tmps);
      |       end
      |     end
      |     if isnan(fltUGain)
      |       if ~strcmp(fltUGain_bkup,'0')
      |         set_param(gcb,'fltUGain','0');
      |       end
      |     else
      |       tmps=num2str(fltUGain);
      |       if ~strcmp(fltUGain_bkup,tmps)
      |         set_param(gcb,'fltUGain',tmps);
      |       end
      |     end
      |     if isnan(fltWIGain)
      |       if ~strcmp(fltWIGain_bkup,'0')
      |         set_param(gcb,'fltWIGain','0');
      |       end
      |     else
      |       tmps=num2str(fltWIGain);
      |       if ~strcmp(fltWIGain_bkup,tmps)
      |         set_param(gcb,'fltWIGain',tmps);
      |       end
      |     end
      |     if isnan(fltEGain)
      |       if ~strcmp(fltEGain_bkup,'0')
      |         set_param(gcb,'fltEGain','0');
      |       end
      |     else
      |       tmps=num2str(fltEGain);
      |       if ~strcmp(fltEGain_bkup,tmps)
      |         set_param(gcb,'fltEGain',tmps);
      |       end
      |     end
      |     if isnan(fltCC1sc_D)
      |       if ~strcmp(fltCC1sc_D_bkup,'0')
      |         set_param(gcb,'fltCC1sc_D','0');
      |       end
      |     else
      |       tmps=num2str(fltCC1sc_D);
      |       if ~strcmp(fltCC1sc_D_bkup,tmps)
      |         set_param(gcb,'fltCC1sc_D',tmps);
      |       end
      |     end
      |     if isnan(fltCC2sc_D)
      |       if ~strcmp(fltCC2sc_D_bkup,'0')
      |         set_param(gcb,'fltCC2sc_D','0');
      |       end
      |     else
      |       tmps=num2str(fltCC2sc_D);
      |       if ~strcmp(fltCC2sc_D_bkup,tmps)
      |         set_param(gcb,'fltCC2sc_D',tmps);
      |       end
      |     end
      |     if isnan(fltUpperLimit_D)
      |       if ~strcmp(fltUpperLimit_D_bkup,'0')
      |         set_param(gcb,'fltUpperLimit_D','0');
      |       end
      |     else
      |       tmps=num2str(fltUpperLimit_D);
      |       if ~strcmp(fltUpperLimit_D_bkup,tmps)
      |         set_param(gcb,'fltUpperLimit_D',tmps);
      |       end
      |     end
      |     if isnan(fltLowerLimit_D)
      |       if ~strcmp(fltLowerLimit_D_bkup,'0')
      |         set_param(gcb,'fltLowerLimit_D','0');
      |       end
      |     else
      |       tmps=num2str(fltLowerLimit_D);
      |       if ~strcmp(fltLowerLimit_D_bkup,tmps)
      |         set_param(gcb,'fltLowerLimit_D',tmps);
      |       end
      |     end
      |     if isnan(fltCC1sc_Q)
      |       if ~strcmp(fltCC1sc_Q_bkup,'0')
      |         set_param(gcb,'fltCC1sc_Q','0');
      |       end
      |     else
      |       tmps=num2str(fltCC1sc_Q);
      |       if ~strcmp(fltCC1sc_Q_bkup,tmps)
      |         set_param(gcb,'fltCC1sc_Q',tmps);
      |       end
      |     end
      |     if isnan(fltCC2sc_Q)
      |       if ~strcmp(fltCC2sc_Q_bkup,'0')
      |         set_param(gcb,'fltCC2sc_Q','0');
      |       end
      |     else
      |       tmps=num2str(fltCC2sc_Q);
      |       if ~strcmp(fltCC2sc_Q_bkup,tmps)
      |         set_param(gcb,'fltCC2sc_Q',tmps);
      |       end
      |     end
      |     if isnan(fltUpperLimit_Q)
      |       if ~strcmp(fltUpperLimit_Q_bkup,'0')
      |         set_param(gcb,'fltUpperLimit_Q','0');
      |       end
      |     else
      |       tmps=num2str(fltUpperLimit_Q);
      |       if ~strcmp(fltUpperLimit_Q_bkup,tmps)
      |         set_param(gcb,'fltUpperLimit_Q',tmps);
      |       end
      |     end
      |     if isnan(fltLowerLimit_Q)
      |       if ~strcmp(fltLowerLimit_Q_bkup,'0')
      |         set_param(gcb,'fltLowerLimit_Q','0');
      |       end
      |     else
      |       tmps=num2str(fltLowerLimit_Q);
      |       if ~strcmp(fltLowerLimit_Q_bkup,tmps)
      |         set_param(gcb,'fltLowerLimit_Q',tmps);
      |       end
      |     end
      |   end
      | end
      mask TypeOptions intmethod: Forward Rectangular | Backward Rectangular | Trapezoidal
      mask Callback intmethod:
      | autoCalcEn=get_param(gcb,'autoCalcEn');
      | if strcmp(autoCalcEn,'on')
      |   SampleTime=Simulink.data.evalinGlobal(bdroot,get_param(gcb,'SampleTime'));
      |   if (SampleTime==-1)
      |     SampleTime=str2double(get_param(gcb,'SampleTime_1'));
      |   end
      |   fltIGain_bkup=get_param(gcb,'fltIGain');
      |   fltUGain_bkup=get_param(gcb,'fltUGain');
      |   fltWIGain_bkup=get_param(gcb,'fltWIGain');
      |   fltEGain_bkup=get_param(gcb,'fltEGain');
      |   fltCC1sc_D_bkup=get_param(gcb,'fltCC1sc_D');
      |   fltCC2sc_D_bkup=get_param(gcb,'fltCC2sc_D');
      |   fltUpperLimit_D_bkup=get_param(gcb,'fltUpperLimit_D');
      |   fltLowerLimit_D_bkup=get_param(gcb,'fltLowerLimit_D');
      |   fltCC1sc_Q_bkup=get_param(gcb,'fltCC1sc_Q');
      |   fltCC2sc_Q_bkup=get_param(gcb,'fltCC2sc_Q');
      |   fltUpperLimit_Q_bkup=get_param(gcb,'fltUpperLimit_Q');
      |   fltLowerLimit_Q_bkup=get_param(gcb,'fltLowerLimit_Q');
      |   intmethod=get_param(gcb,'intmethod');
      |   if0=Simulink.data.evalinGlobal(bdroot,get_param(gcb,'if0'));
      |   iksi=Simulink.data.evalinGlobal(bdroot,get_param(gcb,'iksi'));
      |   Ld=Simulink.data.evalinGlobal(bdroot,get_param(gcb,'Ld'));
      |   Lq=Simulink.data.evalinGlobal(bdroot,get_param(gcb,'Lq'));
      |   Rs=Simulink.data.evalinGlobal(bdroot,get_param(gcb,'Rs'));
      |   mechspeed=Simulink.data.evalinGlobal(bdroot,get_param(gcb,'mechspeed'));
      |   polepairs=Simulink.data.evalinGlobal(bdroot,get_param(gcb,'polepairs'));
      |   if (if0<=0)
      |     warning('Natural frequency f0 must be positive.');
      |   end
      |   if (iksi<=0)
      |     warning('Current loop attenuation must be positive.');
      |   end
      |   if (iksi>1)
      |     warning('Current loop attenuation must not exceed 1.');
      |   end
      |   if (Ld<=0)
      |     warning('Inductance Ld must be positive.');
      |   end
      |   if (Lq<=0)
      |     warning('Inductance Lq must be positive.');
      |   end
      |   if (Rs<0)
      |     warning('Resistance Rs must be non-negative.');
      |   end
      |   if (mechspeed<=0)
      |     warning('Max. speed must be positive.');
      |   end
      |   if (polepairs<1)
      |     warning('Number of pole pairs must be a natural number (1, 2, 3, ...).');
      |   end
      |   if (round(polepairs)~=polepairs)
      |     warning('Number of pole pairs must be a natural number (1, 2, 3, ...).');
      |   end
      |   w0=6.283185307179586*if0;
      |   pgain=2.0*iksi*w0*Ld-Rs;
      |   igain=w0*w0*Ld;
      |   if strcmp(intmethod,'Forward Rectangular')
      |     cc1=pgain;
      |     cc2=-pgain+igain*SampleTime;
      |   else
      |     if strcmp(intmethod,'Backward Rectangular')
      |       cc1=pgain+igain*SampleTime;
      |       cc2=-pgain;
      |     else
      |       cc1=pgain+igain*SampleTime*0.5;
      |       cc2=-pgain+igain*SampleTime*0.5;
      |     end
      |   end
      |   fltCC1sc_D=cc1;
      |   fltCC2sc_D=cc2;
      |   fltCC1sc_Q=fltCC1sc_D;
      |   fltCC2sc_Q=fltCC2sc_D;
      |   fltLowerLimit_D=-1000000.0;
      |   fltUpperLimit_D=1000000.0;
      |   fltLowerLimit_Q=fltLowerLimit_D;
      |   fltUpperLimit_Q=fltUpperLimit_D;
      |   fltIGain=(2.0*Ld-SampleTime*Rs)/(2.0*Ld+SampleTime*Rs);
      |   fltUGain=SampleTime/(2.0*Ld+SampleTime*Rs);
      |   fltWIGain=SampleTime*Lq/(2.0*Ld+SampleTime*Rs);
      |   fltEGain=SampleTime/(2.0*Ld+SampleTime*Rs);
      |   if isnan(fltIGain)
      |     if ~strcmp(fltIGain_bkup,'0')
      |       set_param(gcb,'fltIGain','0');
      |     end
      |   else
      |     tmps=num2str(fltIGain);
      |     if ~strcmp(fltIGain_bkup,tmps)
      |       set_param(gcb,'fltIGain',tmps);
      |     end
      |   end
      |   if isnan(fltUGain)
      |     if ~strcmp(fltUGain_bkup,'0')
      |       set_param(gcb,'fltUGain','0');
      |     end
      |   else
      |     tmps=num2str(fltUGain);
      |     if ~strcmp(fltUGain_bkup,tmps)
      |       set_param(gcb,'fltUGain',tmps);
      |     end
      |   end
      |   if isnan(fltWIGain)
      |     if ~strcmp(fltWIGain_bkup,'0')
      |       set_param(gcb,'fltWIGain','0');
      |     end
      |   else
      |     tmps=num2str(fltWIGain);
      |     if ~strcmp(fltWIGain_bkup,tmps)
      |       set_param(gcb,'fltWIGain',tmps);
      |     end
      |   end
      |   if isnan(fltEGain)
      |     if ~strcmp(fltEGain_bkup,'0')
      |       set_param(gcb,'fltEGain','0');
      |     end
      |   else
      |     tmps=num2str(fltEGain);
      |     if ~strcmp(fltEGain_bkup,tmps)
      |       set_param(gcb,'fltEGain',tmps);
      |     end
      |   end
      |   if isnan(fltCC1sc_D)
      |     if ~strcmp(fltCC1sc_D_bkup,'0')
      |       set_param(gcb,'fltCC1sc_D','0');
      |     end
      |   else
      |     tmps=num2str(fltCC1sc_D);
      |     if ~strcmp(fltCC1sc_D_bkup,tmps)
      |       set_param(gcb,'fltCC1sc_D',tmps);
      |     end
      |   end
      |   if isnan(fltCC2sc_D)
      |     if ~strcmp(fltCC2sc_D_bkup,'0')
      |       set_param(gcb,'fltCC2sc_D','0');
      |     end
      |   else
      |     tmps=num2str(fltCC2sc_D);
      |     if ~strcmp(fltCC2sc_D_bkup,tmps)
      |       set_param(gcb,'fltCC2sc_D',tmps);
      |     end
      |   end
      |   if isnan(fltUpperLimit_D)
      |     if ~strcmp(fltUpperLimit_D_bkup,'0')
      |       set_param(gcb,'fltUpperLimit_D','0');
      |     end
      |   else
      |     tmps=num2str(fltUpperLimit_D);
      |     if ~strcmp(fltUpperLimit_D_bkup,tmps)
      |       set_param(gcb,'fltUpperLimit_D',tmps);
      |     end
      |   end
      |   if isnan(fltLowerLimit_D)
      |     if ~strcmp(fltLowerLimit_D_bkup,'0')
      |       set_param(gcb,'fltLowerLimit_D','0');
      |     end
      |   else
      |     tmps=num2str(fltLowerLimit_D);
      |     if ~strcmp(fltLowerLimit_D_bkup,tmps)
      |       set_param(gcb,'fltLowerLimit_D',tmps);
      |     end
      |   end
      |   if isnan(fltCC1sc_Q)
      |     if ~strcmp(fltCC1sc_Q_bkup,'0')
      |       set_param(gcb,'fltCC1sc_Q','0');
      |     end
      |   else
      |     tmps=num2str(fltCC1sc_Q);
      |     if ~strcmp(fltCC1sc_Q_bkup,tmps)
      |       set_param(gcb,'fltCC1sc_Q',tmps);
      |     end
      |   end
      |   if isnan(fltCC2sc_Q)
      |     if ~strcmp(fltCC2sc_Q_bkup,'0')
      |       set_param(gcb,'fltCC2sc_Q','0');
      |     end
      |   else
      |     tmps=num2str(fltCC2sc_Q);
      |     if ~strcmp(fltCC2sc_Q_bkup,tmps)
      |       set_param(gcb,'fltCC2sc_Q',tmps);
      |     end
      |   end
      |   if isnan(fltUpperLimit_Q)
      |     if ~strcmp(fltUpperLimit_Q_bkup,'0')
      |       set_param(gcb,'fltUpperLimit_Q','0');
      |     end
      |   else
      |     tmps=num2str(fltUpperLimit_Q);
      |     if ~strcmp(fltUpperLimit_Q_bkup,tmps)
      |       set_param(gcb,'fltUpperLimit_Q',tmps);
      |     end
      |   end
      |   if isnan(fltLowerLimit_Q)
      |     if ~strcmp(fltLowerLimit_Q_bkup,'0')
      |       set_param(gcb,'fltLowerLimit_Q','0');
      |     end
      |   else
      |     tmps=num2str(fltLowerLimit_Q);
      |     if ~strcmp(fltLowerLimit_Q_bkup,tmps)
      |       set_param(gcb,'fltLowerLimit_Q',tmps);
      |     end
      |   end
      | end
      mask Callback if0:
      | autoCalcEn=get_param(gcb,'autoCalcEn');
      | if strcmp(autoCalcEn,'on')
      |   SampleTime=Simulink.data.evalinGlobal(bdroot,get_param(gcb,'SampleTime'));
      |   if (SampleTime==-1)
      |     SampleTime=str2double(get_param(gcb,'SampleTime_1'));
      |   end
      |   fltIGain_bkup=get_param(gcb,'fltIGain');
      |   fltUGain_bkup=get_param(gcb,'fltUGain');
      |   fltWIGain_bkup=get_param(gcb,'fltWIGain');
      |   fltEGain_bkup=get_param(gcb,'fltEGain');
      |   fltCC1sc_D_bkup=get_param(gcb,'fltCC1sc_D');
      |   fltCC2sc_D_bkup=get_param(gcb,'fltCC2sc_D');
      |   fltUpperLimit_D_bkup=get_param(gcb,'fltUpperLimit_D');
      |   fltLowerLimit_D_bkup=get_param(gcb,'fltLowerLimit_D');
      |   fltCC1sc_Q_bkup=get_param(gcb,'fltCC1sc_Q');
      |   fltCC2sc_Q_bkup=get_param(gcb,'fltCC2sc_Q');
      |   fltUpperLimit_Q_bkup=get_param(gcb,'fltUpperLimit_Q');
      |   fltLowerLimit_Q_bkup=get_param(gcb,'fltLowerLimit_Q');
      |   intmethod=get_param(gcb,'intmethod');
      |   if0=Simulink.data.evalinGlobal(bdroot,get_param(gcb,'if0'));
      |   iksi=Simulink.data.evalinGlobal(bdroot,get_param(gcb,'iksi'));
      |   Ld=Simulink.data.evalinGlobal(bdroot,get_param(gcb,'Ld'));
      |   Lq=Simulink.data.evalinGlobal(bdroot,get_param(gcb,'Lq'));
      |   Rs=Simulink.data.evalinGlobal(bdroot,get_param(gcb,'Rs'));
      |   mechspeed=Simulink.data.evalinGlobal(bdroot,get_param(gcb,'mechspeed'));
      |   polepairs=Simulink.data.evalinGlobal(bdroot,get_param(gcb,'polepairs'));
      |   if (if0<=0)
      |     warning('Natural frequency f0 must be positive.');
      |   end
      |   if (iksi<=0)
      |     warning('Current loop attenuation must be positive.');
      |   end
      |   if (iksi>1)
      |     warning('Current loop attenuation must not exceed 1.');
      |   end
      |   if (Ld<=0)
      |     warning('Inductance Ld must be positive.');
      |   end
      |   if (Lq<=0)
      |     warning('Inductance Lq must be positive.');
      |   end
      |   if (Rs<0)
      |     warning('Resistance Rs must be non-negative.');
      |   end
      |   if (mechspeed<=0)
      |     warning('Max. speed must be positive.');
      |   end
      |   if (polepairs<1)
      |     warning('Number of pole pairs must be a natural number (1, 2, 3, ...).');
      |   end
      |   if (round(polepairs)~=polepairs)
      |     warning('Number of pole pairs must be a natural number (1, 2, 3, ...).');
      |   end
      |   w0=6.283185307179586*if0;
      |   pgain=2.0*iksi*w0*Ld-Rs;
      |   igain=w0*w0*Ld;
      |   if strcmp(intmethod,'Forward Rectangular')
      |     cc1=pgain;
      |     cc2=-pgain+igain*SampleTime;
      |   else
      |     if strcmp(intmethod,'Backward Rectangular')
      |       cc1=pgain+igain*SampleTime;
      |       cc2=-pgain;
      |     else
      |       cc1=pgain+igain*SampleTime*0.5;
      |       cc2=-pgain+igain*SampleTime*0.5;
      |     end
      |   end
      |   fltCC1sc_D=cc1;
      |   fltCC2sc_D=cc2;
      |   fltCC1sc_Q=fltCC1sc_D;
      |   fltCC2sc_Q=fltCC2sc_D;
      |   fltLowerLimit_D=-1000000.0;
      |   fltUpperLimit_D=1000000.0;
      |   fltLowerLimit_Q=fltLowerLimit_D;
      |   fltUpperLimit_Q=fltUpperLimit_D;
      |   fltIGain=(2.0*Ld-SampleTime*Rs)/(2.0*Ld+SampleTime*Rs);
      |   fltUGain=SampleTime/(2.0*Ld+SampleTime*Rs);
      |   fltWIGain=SampleTime*Lq/(2.0*Ld+SampleTime*Rs);
      |   fltEGain=SampleTime/(2.0*Ld+SampleTime*Rs);
      |   if isnan(fltIGain)
      |     if ~strcmp(fltIGain_bkup,'0')
      |       set_param(gcb,'fltIGain','0');
      |     end
      |   else
      |     tmps=num2str(fltIGain);
      |     if ~strcmp(fltIGain_bkup,tmps)
      |       set_param(gcb,'fltIGain',tmps);
      |     end
      |   end
      |   if isnan(fltUGain)
      |     if ~strcmp(fltUGain_bkup,'0')
      |       set_param(gcb,'fltUGain','0');
      |     end
      |   else
      |     tmps=num2str(fltUGain);
      |     if ~strcmp(fltUGain_bkup,tmps)
      |       set_param(gcb,'fltUGain',tmps);
      |     end
      |   end
      |   if isnan(fltWIGain)
      |     if ~strcmp(fltWIGain_bkup,'0')
      |       set_param(gcb,'fltWIGain','0');
      |     end
      |   else
      |     tmps=num2str(fltWIGain);
      |     if ~strcmp(fltWIGain_bkup,tmps)
      |       set_param(gcb,'fltWIGain',tmps);
      |     end
      |   end
      |   if isnan(fltEGain)
      |     if ~strcmp(fltEGain_bkup,'0')
      |       set_param(gcb,'fltEGain','0');
      |     end
      |   else
      |     tmps=num2str(fltEGain);
      |     if ~strcmp(fltEGain_bkup,tmps)
      |       set_param(gcb,'fltEGain',tmps);
      |     end
      |   end
      |   if isnan(fltCC1sc_D)
      |     if ~strcmp(fltCC1sc_D_bkup,'0')
      |       set_param(gcb,'fltCC1sc_D','0');
      |     end
      |   else
      |     tmps=num2str(fltCC1sc_D);
      |     if ~strcmp(fltCC1sc_D_bkup,tmps)
      |       set_param(gcb,'fltCC1sc_D',tmps);
      |     end
      |   end
      |   if isnan(fltCC2sc_D)
      |     if ~strcmp(fltCC2sc_D_bkup,'0')
      |       set_param(gcb,'fltCC2sc_D','0');
      |     end
      |   else
      |     tmps=num2str(fltCC2sc_D);
      |     if ~strcmp(fltCC2sc_D_bkup,tmps)
      |       set_param(gcb,'fltCC2sc_D',tmps);
      |     end
      |   end
      |   if isnan(fltUpperLimit_D)
      |     if ~strcmp(fltUpperLimit_D_bkup,'0')
      |       set_param(gcb,'fltUpperLimit_D','0');
      |     end
      |   else
      |     tmps=num2str(fltUpperLimit_D);
      |     if ~strcmp(fltUpperLimit_D_bkup,tmps)
      |       set_param(gcb,'fltUpperLimit_D',tmps);
      |     end
      |   end
      |   if isnan(fltLowerLimit_D)
      |     if ~strcmp(fltLowerLimit_D_bkup,'0')
      |       set_param(gcb,'fltLowerLimit_D','0');
      |     end
      |   else
      |     tmps=num2str(fltLowerLimit_D);
      |     if ~strcmp(fltLowerLimit_D_bkup,tmps)
      |       set_param(gcb,'fltLowerLimit_D',tmps);
      |     end
      |   end
      |   if isnan(fltCC1sc_Q)
      |     if ~strcmp(fltCC1sc_Q_bkup,'0')
      |       set_param(gcb,'fltCC1sc_Q','0');
      |     end
      |   else
      |     tmps=num2str(fltCC1sc_Q);
      |     if ~strcmp(fltCC1sc_Q_bkup,tmps)
      |       set_param(gcb,'fltCC1sc_Q',tmps);
      |     end
      |   end
      |   if isnan(fltCC2sc_Q)
      |     if ~strcmp(fltCC2sc_Q_bkup,'0')
      |       set_param(gcb,'fltCC2sc_Q','0');
      |     end
      |   else
      |     tmps=num2str(fltCC2sc_Q);
      |     if ~strcmp(fltCC2sc_Q_bkup,tmps)
      |       set_param(gcb,'fltCC2sc_Q',tmps);
      |     end
      |   end
      |   if isnan(fltUpperLimit_Q)
      |     if ~strcmp(fltUpperLimit_Q_bkup,'0')
      |       set_param(gcb,'fltUpperLimit_Q','0');
      |     end
      |   else
      |     tmps=num2str(fltUpperLimit_Q);
      |     if ~strcmp(fltUpperLimit_Q_bkup,tmps)
      |       set_param(gcb,'fltUpperLimit_Q',tmps);
      |     end
      |   end
      |   if isnan(fltLowerLimit_Q)
      |     if ~strcmp(fltLowerLimit_Q_bkup,'0')
      |       set_param(gcb,'fltLowerLimit_Q','0');
      |     end
      |   else
      |     tmps=num2str(fltLowerLimit_Q);
      |     if ~strcmp(fltLowerLimit_Q_bkup,tmps)
      |       set_param(gcb,'fltLowerLimit_Q',tmps);
      |     end
      |   end
      | end
      mask Callback iksi:
      | autoCalcEn=get_param(gcb,'autoCalcEn');
      | if strcmp(autoCalcEn,'on')
      |   SampleTime=Simulink.data.evalinGlobal(bdroot,get_param(gcb,'SampleTime'));
      |   if (SampleTime==-1)
      |     SampleTime=str2double(get_param(gcb,'SampleTime_1'));
      |   end
      |   fltIGain_bkup=get_param(gcb,'fltIGain');
      |   fltUGain_bkup=get_param(gcb,'fltUGain');
      |   fltWIGain_bkup=get_param(gcb,'fltWIGain');
      |   fltEGain_bkup=get_param(gcb,'fltEGain');
      |   fltCC1sc_D_bkup=get_param(gcb,'fltCC1sc_D');
      |   fltCC2sc_D_bkup=get_param(gcb,'fltCC2sc_D');
      |   fltUpperLimit_D_bkup=get_param(gcb,'fltUpperLimit_D');
      |   fltLowerLimit_D_bkup=get_param(gcb,'fltLowerLimit_D');
      |   fltCC1sc_Q_bkup=get_param(gcb,'fltCC1sc_Q');
      |   fltCC2sc_Q_bkup=get_param(gcb,'fltCC2sc_Q');
      |   fltUpperLimit_Q_bkup=get_param(gcb,'fltUpperLimit_Q');
      |   fltLowerLimit_Q_bkup=get_param(gcb,'fltLowerLimit_Q');
      |   intmethod=get_param(gcb,'intmethod');
      |   if0=Simulink.data.evalinGlobal(bdroot,get_param(gcb,'if0'));
      |   iksi=Simulink.data.evalinGlobal(bdroot,get_param(gcb,'iksi'));
      |   Ld=Simulink.data.evalinGlobal(bdroot,get_param(gcb,'Ld'));
      |   Lq=Simulink.data.evalinGlobal(bdroot,get_param(gcb,'Lq'));
      |   Rs=Simulink.data.evalinGlobal(bdroot,get_param(gcb,'Rs'));
      |   mechspeed=Simulink.data.evalinGlobal(bdroot,get_param(gcb,'mechspeed'));
      |   polepairs=Simulink.data.evalinGlobal(bdroot,get_param(gcb,'polepairs'));
      |   if (if0<=0)
      |     warning('Natural frequency f0 must be positive.');
      |   end
      |   if (iksi<=0)
      |     warning('Current loop attenuation must be positive.');
      |   end
      |   if (iksi>1)
      |     warning('Current loop attenuation must not exceed 1.');
      |   end
      |   if (Ld<=0)
      |     warning('Inductance Ld must be positive.');
      |   end
      |   if (Lq<=0)
      |     warning('Inductance Lq must be positive.');
      |   end
      |   if (Rs<0)
      |     warning('Resistance Rs must be non-negative.');
      |   end
      |   if (mechspeed<=0)
      |     warning('Max. speed must be positive.');
      |   end
      |   if (polepairs<1)
      |     warning('Number of pole pairs must be a natural number (1, 2, 3, ...).');
      |   end
      |   if (round(polepairs)~=polepairs)
      |     warning('Number of pole pairs must be a natural number (1, 2, 3, ...).');
      |   end
      |   w0=6.283185307179586*if0;
      |   pgain=2.0*iksi*w0*Ld-Rs;
      |   igain=w0*w0*Ld;
      |   if strcmp(intmethod,'Forward Rectangular')
      |     cc1=pgain;
      |     cc2=-pgain+igain*SampleTime;
      |   else
      |     if strcmp(intmethod,'Backward Rectangular')
      |       cc1=pgain+igain*SampleTime;
      |       cc2=-pgain;
      |     else
      |       cc1=pgain+igain*SampleTime*0.5;
      |       cc2=-pgain+igain*SampleTime*0.5;
      |     end
      |   end
      |   fltCC1sc_D=cc1;
      |   fltCC2sc_D=cc2;
      |   fltCC1sc_Q=fltCC1sc_D;
      |   fltCC2sc_Q=fltCC2sc_D;
      |   fltLowerLimit_D=-1000000.0;
      |   fltUpperLimit_D=1000000.0;
      |   fltLowerLimit_Q=fltLowerLimit_D;
      |   fltUpperLimit_Q=fltUpperLimit_D;
      |   fltIGain=(2.0*Ld-SampleTime*Rs)/(2.0*Ld+SampleTime*Rs);
      |   fltUGain=SampleTime/(2.0*Ld+SampleTime*Rs);
      |   fltWIGain=SampleTime*Lq/(2.0*Ld+SampleTime*Rs);
      |   fltEGain=SampleTime/(2.0*Ld+SampleTime*Rs);
      |   if isnan(fltIGain)
      |     if ~strcmp(fltIGain_bkup,'0')
      |       set_param(gcb,'fltIGain','0');
      |     end
      |   else
      |     tmps=num2str(fltIGain);
      |     if ~strcmp(fltIGain_bkup,tmps)
      |       set_param(gcb,'fltIGain',tmps);
      |     end
      |   end
      |   if isnan(fltUGain)
      |     if ~strcmp(fltUGain_bkup,'0')
      |       set_param(gcb,'fltUGain','0');
      |     end
      |   else
      |     tmps=num2str(fltUGain);
      |     if ~strcmp(fltUGain_bkup,tmps)
      |       set_param(gcb,'fltUGain',tmps);
      |     end
      |   end
      |   if isnan(fltWIGain)
      |     if ~strcmp(fltWIGain_bkup,'0')
      |       set_param(gcb,'fltWIGain','0');
      |     end
      |   else
      |     tmps=num2str(fltWIGain);
      |     if ~strcmp(fltWIGain_bkup,tmps)
      |       set_param(gcb,'fltWIGain',tmps);
      |     end
      |   end
      |   if isnan(fltEGain)
      |     if ~strcmp(fltEGain_bkup,'0')
      |       set_param(gcb,'fltEGain','0');
      |     end
      |   else
      |     tmps=num2str(fltEGain);
      |     if ~strcmp(fltEGain_bkup,tmps)
      |       set_param(gcb,'fltEGain',tmps);
      |     end
      |   end
      |   if isnan(fltCC1sc_D)
      |     if ~strcmp(fltCC1sc_D_bkup,'0')
      |       set_param(gcb,'fltCC1sc_D','0');
      |     end
      |   else
      |     tmps=num2str(fltCC1sc_D);
      |     if ~strcmp(fltCC1sc_D_bkup,tmps)
      |       set_param(gcb,'fltCC1sc_D',tmps);
      |     end
      |   end
      |   if isnan(fltCC2sc_D)
      |     if ~strcmp(fltCC2sc_D_bkup,'0')
      |       set_param(gcb,'fltCC2sc_D','0');
      |     end
      |   else
      |     tmps=num2str(fltCC2sc_D);
      |     if ~strcmp(fltCC2sc_D_bkup,tmps)
      |       set_param(gcb,'fltCC2sc_D',tmps);
      |     end
      |   end
      |   if isnan(fltUpperLimit_D)
      |     if ~strcmp(fltUpperLimit_D_bkup,'0')
      |       set_param(gcb,'fltUpperLimit_D','0');
      |     end
      |   else
      |     tmps=num2str(fltUpperLimit_D);
      |     if ~strcmp(fltUpperLimit_D_bkup,tmps)
      |       set_param(gcb,'fltUpperLimit_D',tmps);
      |     end
      |   end
      |   if isnan(fltLowerLimit_D)
      |     if ~strcmp(fltLowerLimit_D_bkup,'0')
      |       set_param(gcb,'fltLowerLimit_D','0');
      |     end
      |   else
      |     tmps=num2str(fltLowerLimit_D);
      |     if ~strcmp(fltLowerLimit_D_bkup,tmps)
      |       set_param(gcb,'fltLowerLimit_D',tmps);
      |     end
      |   end
      |   if isnan(fltCC1sc_Q)
      |     if ~strcmp(fltCC1sc_Q_bkup,'0')
      |       set_param(gcb,'fltCC1sc_Q','0');
      |     end
      |   else
      |     tmps=num2str(fltCC1sc_Q);
      |     if ~strcmp(fltCC1sc_Q_bkup,tmps)
      |       set_param(gcb,'fltCC1sc_Q',tmps);
      |     end
      |   end
      |   if isnan(fltCC2sc_Q)
      |     if ~strcmp(fltCC2sc_Q_bkup,'0')
      |       set_param(gcb,'fltCC2sc_Q','0');
      |     end
      |   else
      |     tmps=num2str(fltCC2sc_Q);
      |     if ~strcmp(fltCC2sc_Q_bkup,tmps)
      |       set_param(gcb,'fltCC2sc_Q',tmps);
      |     end
      |   end
      |   if isnan(fltUpperLimit_Q)
      |     if ~strcmp(fltUpperLimit_Q_bkup,'0')
      |       set_param(gcb,'fltUpperLimit_Q','0');
      |     end
      |   else
      |     tmps=num2str(fltUpperLimit_Q);
      |     if ~strcmp(fltUpperLimit_Q_bkup,tmps)
      |       set_param(gcb,'fltUpperLimit_Q',tmps);
      |     end
      |   end
      |   if isnan(fltLowerLimit_Q)
      |     if ~strcmp(fltLowerLimit_Q_bkup,'0')
      |       set_param(gcb,'fltLowerLimit_Q','0');
      |     end
      |   else
      |     tmps=num2str(fltLowerLimit_Q);
      |     if ~strcmp(fltLowerLimit_Q_bkup,tmps)
      |       set_param(gcb,'fltLowerLimit_Q',tmps);
      |     end
      |   end
      | end
      mask Callback Ld:
      | autoCalcEn=get_param(gcb,'autoCalcEn');
      | if strcmp(autoCalcEn,'on')
      |   SampleTime=Simulink.data.evalinGlobal(bdroot,get_param(gcb,'SampleTime'));
      |   if (SampleTime==-1)
      |     SampleTime=str2double(get_param(gcb,'SampleTime_1'));
      |   end
      |   fltIGain_bkup=get_param(gcb,'fltIGain');
      |   fltUGain_bkup=get_param(gcb,'fltUGain');
      |   fltWIGain_bkup=get_param(gcb,'fltWIGain');
      |   fltEGain_bkup=get_param(gcb,'fltEGain');
      |   fltCC1sc_D_bkup=get_param(gcb,'fltCC1sc_D');
      |   fltCC2sc_D_bkup=get_param(gcb,'fltCC2sc_D');
      |   fltUpperLimit_D_bkup=get_param(gcb,'fltUpperLimit_D');
      |   fltLowerLimit_D_bkup=get_param(gcb,'fltLowerLimit_D');
      |   fltCC1sc_Q_bkup=get_param(gcb,'fltCC1sc_Q');
      |   fltCC2sc_Q_bkup=get_param(gcb,'fltCC2sc_Q');
      |   fltUpperLimit_Q_bkup=get_param(gcb,'fltUpperLimit_Q');
      |   fltLowerLimit_Q_bkup=get_param(gcb,'fltLowerLimit_Q');
      |   intmethod=get_param(gcb,'intmethod');
      |   if0=Simulink.data.evalinGlobal(bdroot,get_param(gcb,'if0'));
      |   iksi=Simulink.data.evalinGlobal(bdroot,get_param(gcb,'iksi'));
      |   Ld=Simulink.data.evalinGlobal(bdroot,get_param(gcb,'Ld'));
      |   Lq=Simulink.data.evalinGlobal(bdroot,get_param(gcb,'Lq'));
      |   Rs=Simulink.data.evalinGlobal(bdroot,get_param(gcb,'Rs'));
      |   mechspeed=Simulink.data.evalinGlobal(bdroot,get_param(gcb,'mechspeed'));
      |   polepairs=Simulink.data.evalinGlobal(bdroot,get_param(gcb,'polepairs'));
      |   if (if0<=0)
      |     warning('Natural frequency f0 must be positive.');
      |   end
      |   if (iksi<=0)
      |     warning('Current loop attenuation must be positive.');
      |   end
      |   if (iksi>1)
      |     warning('Current loop attenuation must not exceed 1.');
      |   end
      |   if (Ld<=0)
      |     warning('Inductance Ld must be positive.');
      |   end
      |   if (Lq<=0)
      |     warning('Inductance Lq must be positive.');
      |   end
      |   if (Rs<0)
      |     warning('Resistance Rs must be non-negative.');
      |   end
      |   if (mechspeed<=0)
      |     warning('Max. speed must be positive.');
      |   end
      |   if (polepairs<1)
      |     warning('Number of pole pairs must be a natural number (1, 2, 3, ...).');
      |   end
      |   if (round(polepairs)~=polepairs)
      |     warning('Number of pole pairs must be a natural number (1, 2, 3, ...).');
      |   end
      |   w0=6.283185307179586*if0;
      |   pgain=2.0*iksi*w0*Ld-Rs;
      |   igain=w0*w0*Ld;
      |   if strcmp(intmethod,'Forward Rectangular')
      |     cc1=pgain;
      |     cc2=-pgain+igain*SampleTime;
      |   else
      |     if strcmp(intmethod,'Backward Rectangular')
      |       cc1=pgain+igain*SampleTime;
      |       cc2=-pgain;
      |     else
      |       cc1=pgain+igain*SampleTime*0.5;
      |       cc2=-pgain+igain*SampleTime*0.5;
      |     end
      |   end
      |   fltCC1sc_D=cc1;
      |   fltCC2sc_D=cc2;
      |   fltCC1sc_Q=fltCC1sc_D;
      |   fltCC2sc_Q=fltCC2sc_D;
      |   fltLowerLimit_D=-1000000.0;
      |   fltUpperLimit_D=1000000.0;
      |   fltLowerLimit_Q=fltLowerLimit_D;
      |   fltUpperLimit_Q=fltUpperLimit_D;
      |   fltIGain=(2.0*Ld-SampleTime*Rs)/(2.0*Ld+SampleTime*Rs);
      |   fltUGain=SampleTime/(2.0*Ld+SampleTime*Rs);
      |   fltWIGain=SampleTime*Lq/(2.0*Ld+SampleTime*Rs);
      |   fltEGain=SampleTime/(2.0*Ld+SampleTime*Rs);
      |   if isnan(fltIGain)
      |     if ~strcmp(fltIGain_bkup,'0')
      |       set_param(gcb,'fltIGain','0');
      |     end
      |   else
      |     tmps=num2str(fltIGain);
      |     if ~strcmp(fltIGain_bkup,tmps)
      |       set_param(gcb,'fltIGain',tmps);
      |     end
      |   end
      |   if isnan(fltUGain)
      |     if ~strcmp(fltUGain_bkup,'0')
      |       set_param(gcb,'fltUGain','0');
      |     end
      |   else
      |     tmps=num2str(fltUGain);
      |     if ~strcmp(fltUGain_bkup,tmps)
      |       set_param(gcb,'fltUGain',tmps);
      |     end
      |   end
      |   if isnan(fltWIGain)
      |     if ~strcmp(fltWIGain_bkup,'0')
      |       set_param(gcb,'fltWIGain','0');
      |     end
      |   else
      |     tmps=num2str(fltWIGain);
      |     if ~strcmp(fltWIGain_bkup,tmps)
      |       set_param(gcb,'fltWIGain',tmps);
      |     end
      |   end
      |   if isnan(fltEGain)
      |     if ~strcmp(fltEGain_bkup,'0')
      |       set_param(gcb,'fltEGain','0');
      |     end
      |   else
      |     tmps=num2str(fltEGain);
      |     if ~strcmp(fltEGain_bkup,tmps)
      |       set_param(gcb,'fltEGain',tmps);
      |     end
      |   end
      |   if isnan(fltCC1sc_D)
      |     if ~strcmp(fltCC1sc_D_bkup,'0')
      |       set_param(gcb,'fltCC1sc_D','0');
      |     end
      |   else
      |     tmps=num2str(fltCC1sc_D);
      |     if ~strcmp(fltCC1sc_D_bkup,tmps)
      |       set_param(gcb,'fltCC1sc_D',tmps);
      |     end
      |   end
      |   if isnan(fltCC2sc_D)
      |     if ~strcmp(fltCC2sc_D_bkup,'0')
      |       set_param(gcb,'fltCC2sc_D','0');
      |     end
      |   else
      |     tmps=num2str(fltCC2sc_D);
      |     if ~strcmp(fltCC2sc_D_bkup,tmps)
      |       set_param(gcb,'fltCC2sc_D',tmps);
      |     end
      |   end
      |   if isnan(fltUpperLimit_D)
      |     if ~strcmp(fltUpperLimit_D_bkup,'0')
      |       set_param(gcb,'fltUpperLimit_D','0');
      |     end
      |   else
      |     tmps=num2str(fltUpperLimit_D);
      |     if ~strcmp(fltUpperLimit_D_bkup,tmps)
      |       set_param(gcb,'fltUpperLimit_D',tmps);
      |     end
      |   end
      |   if isnan(fltLowerLimit_D)
      |     if ~strcmp(fltLowerLimit_D_bkup,'0')
      |       set_param(gcb,'fltLowerLimit_D','0');
      |     end
      |   else
      |     tmps=num2str(fltLowerLimit_D);
      |     if ~strcmp(fltLowerLimit_D_bkup,tmps)
      |       set_param(gcb,'fltLowerLimit_D',tmps);
      |     end
      |   end
      |   if isnan(fltCC1sc_Q)
      |     if ~strcmp(fltCC1sc_Q_bkup,'0')
      |       set_param(gcb,'fltCC1sc_Q','0');
      |     end
      |   else
      |     tmps=num2str(fltCC1sc_Q);
      |     if ~strcmp(fltCC1sc_Q_bkup,tmps)
      |       set_param(gcb,'fltCC1sc_Q',tmps);
      |     end
      |   end
      |   if isnan(fltCC2sc_Q)
      |     if ~strcmp(fltCC2sc_Q_bkup,'0')
      |       set_param(gcb,'fltCC2sc_Q','0');
      |     end
      |   else
      |     tmps=num2str(fltCC2sc_Q);
      |     if ~strcmp(fltCC2sc_Q_bkup,tmps)
      |       set_param(gcb,'fltCC2sc_Q',tmps);
      |     end
      |   end
      |   if isnan(fltUpperLimit_Q)
      |     if ~strcmp(fltUpperLimit_Q_bkup,'0')
      |       set_param(gcb,'fltUpperLimit_Q','0');
      |     end
      |   else
      |     tmps=num2str(fltUpperLimit_Q);
      |     if ~strcmp(fltUpperLimit_Q_bkup,tmps)
      |       set_param(gcb,'fltUpperLimit_Q',tmps);
      |     end
      |   end
      |   if isnan(fltLowerLimit_Q)
      |     if ~strcmp(fltLowerLimit_Q_bkup,'0')
      |       set_param(gcb,'fltLowerLimit_Q','0');
      |     end
      |   else
      |     tmps=num2str(fltLowerLimit_Q);
      |     if ~strcmp(fltLowerLimit_Q_bkup,tmps)
      |       set_param(gcb,'fltLowerLimit_Q',tmps);
      |     end
      |   end
      | end
      mask Callback Lq:
      | autoCalcEn=get_param(gcb,'autoCalcEn');
      | if strcmp(autoCalcEn,'on')
      |   SampleTime=Simulink.data.evalinGlobal(bdroot,get_param(gcb,'SampleTime'));
      |   if (SampleTime==-1)
      |     SampleTime=str2double(get_param(gcb,'SampleTime_1'));
      |   end
      |   fltIGain_bkup=get_param(gcb,'fltIGain');
      |   fltUGain_bkup=get_param(gcb,'fltUGain');
      |   fltWIGain_bkup=get_param(gcb,'fltWIGain');
      |   fltEGain_bkup=get_param(gcb,'fltEGain');
      |   fltCC1sc_D_bkup=get_param(gcb,'fltCC1sc_D');
      |   fltCC2sc_D_bkup=get_param(gcb,'fltCC2sc_D');
      |   fltUpperLimit_D_bkup=get_param(gcb,'fltUpperLimit_D');
      |   fltLowerLimit_D_bkup=get_param(gcb,'fltLowerLimit_D');
      |   fltCC1sc_Q_bkup=get_param(gcb,'fltCC1sc_Q');
      |   fltCC2sc_Q_bkup=get_param(gcb,'fltCC2sc_Q');
      |   fltUpperLimit_Q_bkup=get_param(gcb,'fltUpperLimit_Q');
      |   fltLowerLimit_Q_bkup=get_param(gcb,'fltLowerLimit_Q');
      |   intmethod=get_param(gcb,'intmethod');
      |   if0=Simulink.data.evalinGlobal(bdroot,get_param(gcb,'if0'));
      |   iksi=Simulink.data.evalinGlobal(bdroot,get_param(gcb,'iksi'));
      |   Ld=Simulink.data.evalinGlobal(bdroot,get_param(gcb,'Ld'));
      |   Lq=Simulink.data.evalinGlobal(bdroot,get_param(gcb,'Lq'));
      |   Rs=Simulink.data.evalinGlobal(bdroot,get_param(gcb,'Rs'));
      |   mechspeed=Simulink.data.evalinGlobal(bdroot,get_param(gcb,'mechspeed'));
      |   polepairs=Simulink.data.evalinGlobal(bdroot,get_param(gcb,'polepairs'));
      |   if (if0<=0)
      |     warning('Natural frequency f0 must be positive.');
      |   end
      |   if (iksi<=0)
      |     warning('Current loop attenuation must be positive.');
      |   end
      |   if (iksi>1)
      |     warning('Current loop attenuation must not exceed 1.');
      |   end
      |   if (Ld<=0)
      |     warning('Inductance Ld must be positive.');
      |   end
      |   if (Lq<=0)
      |     warning('Inductance Lq must be positive.');
      |   end
      |   if (Rs<0)
      |     warning('Resistance Rs must be non-negative.');
      |   end
      |   if (mechspeed<=0)
      |     warning('Max. speed must be positive.');
      |   end
      |   if (polepairs<1)
      |     warning('Number of pole pairs must be a natural number (1, 2, 3, ...).');
      |   end
      |   if (round(polepairs)~=polepairs)
      |     warning('Number of pole pairs must be a natural number (1, 2, 3, ...).');
      |   end
      |   w0=6.283185307179586*if0;
      |   pgain=2.0*iksi*w0*Ld-Rs;
      |   igain=w0*w0*Ld;
      |   if strcmp(intmethod,'Forward Rectangular')
      |     cc1=pgain;
      |     cc2=-pgain+igain*SampleTime;
      |   else
      |     if strcmp(intmethod,'Backward Rectangular')
      |       cc1=pgain+igain*SampleTime;
      |       cc2=-pgain;
      |     else
      |       cc1=pgain+igain*SampleTime*0.5;
      |       cc2=-pgain+igain*SampleTime*0.5;
      |     end
      |   end
      |   fltCC1sc_D=cc1;
      |   fltCC2sc_D=cc2;
      |   fltCC1sc_Q=fltCC1sc_D;
      |   fltCC2sc_Q=fltCC2sc_D;
      |   fltLowerLimit_D=-1000000.0;
      |   fltUpperLimit_D=1000000.0;
      |   fltLowerLimit_Q=fltLowerLimit_D;
      |   fltUpperLimit_Q=fltUpperLimit_D;
      |   fltIGain=(2.0*Ld-SampleTime*Rs)/(2.0*Ld+SampleTime*Rs);
      |   fltUGain=SampleTime/(2.0*Ld+SampleTime*Rs);
      |   fltWIGain=SampleTime*Lq/(2.0*Ld+SampleTime*Rs);
      |   fltEGain=SampleTime/(2.0*Ld+SampleTime*Rs);
      |   if isnan(fltIGain)
      |     if ~strcmp(fltIGain_bkup,'0')
      |       set_param(gcb,'fltIGain','0');
      |     end
      |   else
      |     tmps=num2str(fltIGain);
      |     if ~strcmp(fltIGain_bkup,tmps)
      |       set_param(gcb,'fltIGain',tmps);
      |     end
      |   end
      |   if isnan(fltUGain)
      |     if ~strcmp(fltUGain_bkup,'0')
      |       set_param(gcb,'fltUGain','0');
      |     end
      |   else
      |     tmps=num2str(fltUGain);
      |     if ~strcmp(fltUGain_bkup,tmps)
      |       set_param(gcb,'fltUGain',tmps);
      |     end
      |   end
      |   if isnan(fltWIGain)
      |     if ~strcmp(fltWIGain_bkup,'0')
      |       set_param(gcb,'fltWIGain','0');
      |     end
      |   else
      |     tmps=num2str(fltWIGain);
      |     if ~strcmp(fltWIGain_bkup,tmps)
      |       set_param(gcb,'fltWIGain',tmps);
      |     end
      |   end
      |   if isnan(fltEGain)
      |     if ~strcmp(fltEGain_bkup,'0')
      |       set_param(gcb,'fltEGain','0');
      |     end
      |   else
      |     tmps=num2str(fltEGain);
      |     if ~strcmp(fltEGain_bkup,tmps)
      |       set_param(gcb,'fltEGain',tmps);
      |     end
      |   end
      |   if isnan(fltCC1sc_D)
      |     if ~strcmp(fltCC1sc_D_bkup,'0')
      |       set_param(gcb,'fltCC1sc_D','0');
      |     end
      |   else
      |     tmps=num2str(fltCC1sc_D);
      |     if ~strcmp(fltCC1sc_D_bkup,tmps)
      |       set_param(gcb,'fltCC1sc_D',tmps);
      |     end
      |   end
      |   if isnan(fltCC2sc_D)
      |     if ~strcmp(fltCC2sc_D_bkup,'0')
      |       set_param(gcb,'fltCC2sc_D','0');
      |     end
      |   else
      |     tmps=num2str(fltCC2sc_D);
      |     if ~strcmp(fltCC2sc_D_bkup,tmps)
      |       set_param(gcb,'fltCC2sc_D',tmps);
      |     end
      |   end
      |   if isnan(fltUpperLimit_D)
      |     if ~strcmp(fltUpperLimit_D_bkup,'0')
      |       set_param(gcb,'fltUpperLimit_D','0');
      |     end
      |   else
      |     tmps=num2str(fltUpperLimit_D);
      |     if ~strcmp(fltUpperLimit_D_bkup,tmps)
      |       set_param(gcb,'fltUpperLimit_D',tmps);
      |     end
      |   end
      |   if isnan(fltLowerLimit_D)
      |     if ~strcmp(fltLowerLimit_D_bkup,'0')
      |       set_param(gcb,'fltLowerLimit_D','0');
      |     end
      |   else
      |     tmps=num2str(fltLowerLimit_D);
      |     if ~strcmp(fltLowerLimit_D_bkup,tmps)
      |       set_param(gcb,'fltLowerLimit_D',tmps);
      |     end
      |   end
      |   if isnan(fltCC1sc_Q)
      |     if ~strcmp(fltCC1sc_Q_bkup,'0')
      |       set_param(gcb,'fltCC1sc_Q','0');
      |     end
      |   else
      |     tmps=num2str(fltCC1sc_Q);
      |     if ~strcmp(fltCC1sc_Q_bkup,tmps)
      |       set_param(gcb,'fltCC1sc_Q',tmps);
      |     end
      |   end
      |   if isnan(fltCC2sc_Q)
      |     if ~strcmp(fltCC2sc_Q_bkup,'0')
      |       set_param(gcb,'fltCC2sc_Q','0');
      |     end
      |   else
      |     tmps=num2str(fltCC2sc_Q);
      |     if ~strcmp(fltCC2sc_Q_bkup,tmps)
      |       set_param(gcb,'fltCC2sc_Q',tmps);
      |     end
      |   end
      |   if isnan(fltUpperLimit_Q)
      |     if ~strcmp(fltUpperLimit_Q_bkup,'0')
      |       set_param(gcb,'fltUpperLimit_Q','0');
      |     end
      |   else
      |     tmps=num2str(fltUpperLimit_Q);
      |     if ~strcmp(fltUpperLimit_Q_bkup,tmps)
      |       set_param(gcb,'fltUpperLimit_Q',tmps);
      |     end
      |   end
      |   if isnan(fltLowerLimit_Q)
      |     if ~strcmp(fltLowerLimit_Q_bkup,'0')
      |       set_param(gcb,'fltLowerLimit_Q','0');
      |     end
      |   else
      |     tmps=num2str(fltLowerLimit_Q);
      |     if ~strcmp(fltLowerLimit_Q_bkup,tmps)
      |       set_param(gcb,'fltLowerLimit_Q',tmps);
      |     end
      |   end
      | end
      mask Callback Rs:
      | autoCalcEn=get_param(gcb,'autoCalcEn');
      | if strcmp(autoCalcEn,'on')
      |   SampleTime=Simulink.data.evalinGlobal(bdroot,get_param(gcb,'SampleTime'));
      |   if (SampleTime==-1)
      |     SampleTime=str2double(get_param(gcb,'SampleTime_1'));
      |   end
      |   fltIGain_bkup=get_param(gcb,'fltIGain');
      |   fltUGain_bkup=get_param(gcb,'fltUGain');
      |   fltWIGain_bkup=get_param(gcb,'fltWIGain');
      |   fltEGain_bkup=get_param(gcb,'fltEGain');
      |   fltCC1sc_D_bkup=get_param(gcb,'fltCC1sc_D');
      |   fltCC2sc_D_bkup=get_param(gcb,'fltCC2sc_D');
      |   fltUpperLimit_D_bkup=get_param(gcb,'fltUpperLimit_D');
      |   fltLowerLimit_D_bkup=get_param(gcb,'fltLowerLimit_D');
      |   fltCC1sc_Q_bkup=get_param(gcb,'fltCC1sc_Q');
      |   fltCC2sc_Q_bkup=get_param(gcb,'fltCC2sc_Q');
      |   fltUpperLimit_Q_bkup=get_param(gcb,'fltUpperLimit_Q');
      |   fltLowerLimit_Q_bkup=get_param(gcb,'fltLowerLimit_Q');
      |   intmethod=get_param(gcb,'intmethod');
      |   if0=Simulink.data.evalinGlobal(bdroot,get_param(gcb,'if0'));
      |   iksi=Simulink.data.evalinGlobal(bdroot,get_param(gcb,'iksi'));
      |   Ld=Simulink.data.evalinGlobal(bdroot,get_param(gcb,'Ld'));
      |   Lq=Simulink.data.evalinGlobal(bdroot,get_param(gcb,'Lq'));
      |   Rs=Simulink.data.evalinGlobal(bdroot,get_param(gcb,'Rs'));
      |   mechspeed=Simulink.data.evalinGlobal(bdroot,get_param(gcb,'mechspeed'));
      |   polepairs=Simulink.data.evalinGlobal(bdroot,get_param(gcb,'polepairs'));
      |   if (if0<=0)
      |     warning('Natural frequency f0 must be positive.');
      |   end
      |   if (iksi<=0)
      |     warning('Current loop attenuation must be positive.');
      |   end
      |   if (iksi>1)
      |     warning('Current loop attenuation must not exceed 1.');
      |   end
      |   if (Ld<=0)
      |     warning('Inductance Ld must be positive.');
      |   end
      |   if (Lq<=0)
      |     warning('Inductance Lq must be positive.');
      |   end
      |   if (Rs<0)
      |     warning('Resistance Rs must be non-negative.');
      |   end
      |   if (mechspeed<=0)
      |     warning('Max. speed must be positive.');
      |   end
      |   if (polepairs<1)
      |     warning('Number of pole pairs must be a natural number (1, 2, 3, ...).');
      |   end
      |   if (round(polepairs)~=polepairs)
      |     warning('Number of pole pairs must be a natural number (1, 2, 3, ...).');
      |   end
      |   w0=6.283185307179586*if0;
      |   pgain=2.0*iksi*w0*Ld-Rs;
      |   igain=w0*w0*Ld;
      |   if strcmp(intmethod,'Forward Rectangular')
      |     cc1=pgain;
      |     cc2=-pgain+igain*SampleTime;
      |   else
      |     if strcmp(intmethod,'Backward Rectangular')
      |       cc1=pgain+igain*SampleTime;
      |       cc2=-pgain;
      |     else
      |       cc1=pgain+igain*SampleTime*0.5;
      |       cc2=-pgain+igain*SampleTime*0.5;
      |     end
      |   end
      |   fltCC1sc_D=cc1;
      |   fltCC2sc_D=cc2;
      |   fltCC1sc_Q=fltCC1sc_D;
      |   fltCC2sc_Q=fltCC2sc_D;
      |   fltLowerLimit_D=-1000000.0;
      |   fltUpperLimit_D=1000000.0;
      |   fltLowerLimit_Q=fltLowerLimit_D;
      |   fltUpperLimit_Q=fltUpperLimit_D;
      |   fltIGain=(2.0*Ld-SampleTime*Rs)/(2.0*Ld+SampleTime*Rs);
      |   fltUGain=SampleTime/(2.0*Ld+SampleTime*Rs);
      |   fltWIGain=SampleTime*Lq/(2.0*Ld+SampleTime*Rs);
      |   fltEGain=SampleTime/(2.0*Ld+SampleTime*Rs);
      |   if isnan(fltIGain)
      |     if ~strcmp(fltIGain_bkup,'0')
      |       set_param(gcb,'fltIGain','0');
      |     end
      |   else
      |     tmps=num2str(fltIGain);
      |     if ~strcmp(fltIGain_bkup,tmps)
      |       set_param(gcb,'fltIGain',tmps);
      |     end
      |   end
      |   if isnan(fltUGain)
      |     if ~strcmp(fltUGain_bkup,'0')
      |       set_param(gcb,'fltUGain','0');
      |     end
      |   else
      |     tmps=num2str(fltUGain);
      |     if ~strcmp(fltUGain_bkup,tmps)
      |       set_param(gcb,'fltUGain',tmps);
      |     end
      |   end
      |   if isnan(fltWIGain)
      |     if ~strcmp(fltWIGain_bkup,'0')
      |       set_param(gcb,'fltWIGain','0');
      |     end
      |   else
      |     tmps=num2str(fltWIGain);
      |     if ~strcmp(fltWIGain_bkup,tmps)
      |       set_param(gcb,'fltWIGain',tmps);
      |     end
      |   end
      |   if isnan(fltEGain)
      |     if ~strcmp(fltEGain_bkup,'0')
      |       set_param(gcb,'fltEGain','0');
      |     end
      |   else
      |     tmps=num2str(fltEGain);
      |     if ~strcmp(fltEGain_bkup,tmps)
      |       set_param(gcb,'fltEGain',tmps);
      |     end
      |   end
      |   if isnan(fltCC1sc_D)
      |     if ~strcmp(fltCC1sc_D_bkup,'0')
      |       set_param(gcb,'fltCC1sc_D','0');
      |     end
      |   else
      |     tmps=num2str(fltCC1sc_D);
      |     if ~strcmp(fltCC1sc_D_bkup,tmps)
      |       set_param(gcb,'fltCC1sc_D',tmps);
      |     end
      |   end
      |   if isnan(fltCC2sc_D)
      |     if ~strcmp(fltCC2sc_D_bkup,'0')
      |       set_param(gcb,'fltCC2sc_D','0');
      |     end
      |   else
      |     tmps=num2str(fltCC2sc_D);
      |     if ~strcmp(fltCC2sc_D_bkup,tmps)
      |       set_param(gcb,'fltCC2sc_D',tmps);
      |     end
      |   end
      |   if isnan(fltUpperLimit_D)
      |     if ~strcmp(fltUpperLimit_D_bkup,'0')
      |       set_param(gcb,'fltUpperLimit_D','0');
      |     end
      |   else
      |     tmps=num2str(fltUpperLimit_D);
      |     if ~strcmp(fltUpperLimit_D_bkup,tmps)
      |       set_param(gcb,'fltUpperLimit_D',tmps);
      |     end
      |   end
      |   if isnan(fltLowerLimit_D)
      |     if ~strcmp(fltLowerLimit_D_bkup,'0')
      |       set_param(gcb,'fltLowerLimit_D','0');
      |     end
      |   else
      |     tmps=num2str(fltLowerLimit_D);
      |     if ~strcmp(fltLowerLimit_D_bkup,tmps)
      |       set_param(gcb,'fltLowerLimit_D',tmps);
      |     end
      |   end
      |   if isnan(fltCC1sc_Q)
      |     if ~strcmp(fltCC1sc_Q_bkup,'0')
      |       set_param(gcb,'fltCC1sc_Q','0');
      |     end
      |   else
      |     tmps=num2str(fltCC1sc_Q);
      |     if ~strcmp(fltCC1sc_Q_bkup,tmps)
      |       set_param(gcb,'fltCC1sc_Q',tmps);
      |     end
      |   end
      |   if isnan(fltCC2sc_Q)
      |     if ~strcmp(fltCC2sc_Q_bkup,'0')
      |       set_param(gcb,'fltCC2sc_Q','0');
      |     end
      |   else
      |     tmps=num2str(fltCC2sc_Q);
      |     if ~strcmp(fltCC2sc_Q_bkup,tmps)
      |       set_param(gcb,'fltCC2sc_Q',tmps);
      |     end
      |   end
      |   if isnan(fltUpperLimit_Q)
      |     if ~strcmp(fltUpperLimit_Q_bkup,'0')
      |       set_param(gcb,'fltUpperLimit_Q','0');
      |     end
      |   else
      |     tmps=num2str(fltUpperLimit_Q);
      |     if ~strcmp(fltUpperLimit_Q_bkup,tmps)
      |       set_param(gcb,'fltUpperLimit_Q',tmps);
      |     end
      |   end
      |   if isnan(fltLowerLimit_Q)
      |     if ~strcmp(fltLowerLimit_Q_bkup,'0')
      |       set_param(gcb,'fltLowerLimit_Q','0');
      |     end
      |   else
      |     tmps=num2str(fltLowerLimit_Q);
      |     if ~strcmp(fltLowerLimit_Q_bkup,tmps)
      |       set_param(gcb,'fltLowerLimit_Q',tmps);
      |     end
      |   end
      | end
      mask Callback mechspeed:
      | autoCalcEn=get_param(gcb,'autoCalcEn');
      | if strcmp(autoCalcEn,'on')
      |   SampleTime=Simulink.data.evalinGlobal(bdroot,get_param(gcb,'SampleTime'));
      |   if (SampleTime==-1)
      |     SampleTime=str2double(get_param(gcb,'SampleTime_1'));
      |   end
      |   fltIGain_bkup=get_param(gcb,'fltIGain');
      |   fltUGain_bkup=get_param(gcb,'fltUGain');
      |   fltWIGain_bkup=get_param(gcb,'fltWIGain');
      |   fltEGain_bkup=get_param(gcb,'fltEGain');
      |   fltCC1sc_D_bkup=get_param(gcb,'fltCC1sc_D');
      |   fltCC2sc_D_bkup=get_param(gcb,'fltCC2sc_D');
      |   fltUpperLimit_D_bkup=get_param(gcb,'fltUpperLimit_D');
      |   fltLowerLimit_D_bkup=get_param(gcb,'fltLowerLimit_D');
      |   fltCC1sc_Q_bkup=get_param(gcb,'fltCC1sc_Q');
      |   fltCC2sc_Q_bkup=get_param(gcb,'fltCC2sc_Q');
      |   fltUpperLimit_Q_bkup=get_param(gcb,'fltUpperLimit_Q');
      |   fltLowerLimit_Q_bkup=get_param(gcb,'fltLowerLimit_Q');
      |   intmethod=get_param(gcb,'intmethod');
      |   if0=Simulink.data.evalinGlobal(bdroot,get_param(gcb,'if0'));
      |   iksi=Simulink.data.evalinGlobal(bdroot,get_param(gcb,'iksi'));
      |   Ld=Simulink.data.evalinGlobal(bdroot,get_param(gcb,'Ld'));
      |   Lq=Simulink.data.evalinGlobal(bdroot,get_param(gcb,'Lq'));
      |   Rs=Simulink.data.evalinGlobal(bdroot,get_param(gcb,'Rs'));
      |   mechspeed=Simulink.data.evalinGlobal(bdroot,get_param(gcb,'mechspeed'));
      |   polepairs=Simulink.data.evalinGlobal(bdroot,get_param(gcb,'polepairs'));
      |   if (if0<=0)
      |     warning('Natural frequency f0 must be positive.');
      |   end
      |   if (iksi<=0)
      |     warning('Current loop attenuation must be positive.');
      |   end
      |   if (iksi>1)
      |     warning('Current loop attenuation must not exceed 1.');
      |   end
      |   if (Ld<=0)
      |     warning('Inductance Ld must be positive.');
      |   end
      |   if (Lq<=0)
      |     warning('Inductance Lq must be positive.');
      |   end
      |   if (Rs<0)
      |     warning('Resistance Rs must be non-negative.');
      |   end
      |   if (mechspeed<=0)
      |     warning('Max. speed must be positive.');
      |   end
      |   if (polepairs<1)
      |     warning('Number of pole pairs must be a natural number (1, 2, 3, ...).');
      |   end
      |   if (round(polepairs)~=polepairs)
      |     warning('Number of pole pairs must be a natural number (1, 2, 3, ...).');
      |   end
      |   w0=6.283185307179586*if0;
      |   pgain=2.0*iksi*w0*Ld-Rs;
      |   igain=w0*w0*Ld;
      |   if strcmp(intmethod,'Forward Rectangular')
      |     cc1=pgain;
      |     cc2=-pgain+igain*SampleTime;
      |   else
      |     if strcmp(intmethod,'Backward Rectangular')
      |       cc1=pgain+igain*SampleTime;
      |       cc2=-pgain;
      |     else
      |       cc1=pgain+igain*SampleTime*0.5;
      |       cc2=-pgain+igain*SampleTime*0.5;
      |     end
      |   end
      |   fltCC1sc_D=cc1;
      |   fltCC2sc_D=cc2;
      |   fltCC1sc_Q=fltCC1sc_D;
      |   fltCC2sc_Q=fltCC2sc_D;
      |   fltLowerLimit_D=-1000000.0;
      |   fltUpperLimit_D=1000000.0;
      |   fltLowerLimit_Q=fltLowerLimit_D;
      |   fltUpperLimit_Q=fltUpperLimit_D;
      |   fltIGain=(2.0*Ld-SampleTime*Rs)/(2.0*Ld+SampleTime*Rs);
      |   fltUGain=SampleTime/(2.0*Ld+SampleTime*Rs);
      |   fltWIGain=SampleTime*Lq/(2.0*Ld+SampleTime*Rs);
      |   fltEGain=SampleTime/(2.0*Ld+SampleTime*Rs);
      |   if isnan(fltIGain)
      |     if ~strcmp(fltIGain_bkup,'0')
      |       set_param(gcb,'fltIGain','0');
      |     end
      |   else
      |     tmps=num2str(fltIGain);
      |     if ~strcmp(fltIGain_bkup,tmps)
      |       set_param(gcb,'fltIGain',tmps);
      |     end
      |   end
      |   if isnan(fltUGain)
      |     if ~strcmp(fltUGain_bkup,'0')
      |       set_param(gcb,'fltUGain','0');
      |     end
      |   else
      |     tmps=num2str(fltUGain);
      |     if ~strcmp(fltUGain_bkup,tmps)
      |       set_param(gcb,'fltUGain',tmps);
      |     end
      |   end
      |   if isnan(fltWIGain)
      |     if ~strcmp(fltWIGain_bkup,'0')
      |       set_param(gcb,'fltWIGain','0');
      |     end
      |   else
      |     tmps=num2str(fltWIGain);
      |     if ~strcmp(fltWIGain_bkup,tmps)
      |       set_param(gcb,'fltWIGain',tmps);
      |     end
      |   end
      |   if isnan(fltEGain)
      |     if ~strcmp(fltEGain_bkup,'0')
      |       set_param(gcb,'fltEGain','0');
      |     end
      |   else
      |     tmps=num2str(fltEGain);
      |     if ~strcmp(fltEGain_bkup,tmps)
      |       set_param(gcb,'fltEGain',tmps);
      |     end
      |   end
      |   if isnan(fltCC1sc_D)
      |     if ~strcmp(fltCC1sc_D_bkup,'0')
      |       set_param(gcb,'fltCC1sc_D','0');
      |     end
      |   else
      |     tmps=num2str(fltCC1sc_D);
      |     if ~strcmp(fltCC1sc_D_bkup,tmps)
      |       set_param(gcb,'fltCC1sc_D',tmps);
      |     end
      |   end
      |   if isnan(fltCC2sc_D)
      |     if ~strcmp(fltCC2sc_D_bkup,'0')
      |       set_param(gcb,'fltCC2sc_D','0');
      |     end
      |   else
      |     tmps=num2str(fltCC2sc_D);
      |     if ~strcmp(fltCC2sc_D_bkup,tmps)
      |       set_param(gcb,'fltCC2sc_D',tmps);
      |     end
      |   end
      |   if isnan(fltUpperLimit_D)
      |     if ~strcmp(fltUpperLimit_D_bkup,'0')
      |       set_param(gcb,'fltUpperLimit_D','0');
      |     end
      |   else
      |     tmps=num2str(fltUpperLimit_D);
      |     if ~strcmp(fltUpperLimit_D_bkup,tmps)
      |       set_param(gcb,'fltUpperLimit_D',tmps);
      |     end
      |   end
      |   if isnan(fltLowerLimit_D)
      |     if ~strcmp(fltLowerLimit_D_bkup,'0')
      |       set_param(gcb,'fltLowerLimit_D','0');
      |     end
      |   else
      |     tmps=num2str(fltLowerLimit_D);
      |     if ~strcmp(fltLowerLimit_D_bkup,tmps)
      |       set_param(gcb,'fltLowerLimit_D',tmps);
      |     end
      |   end
      |   if isnan(fltCC1sc_Q)
      |     if ~strcmp(fltCC1sc_Q_bkup,'0')
      |       set_param(gcb,'fltCC1sc_Q','0');
      |     end
      |   else
      |     tmps=num2str(fltCC1sc_Q);
      |     if ~strcmp(fltCC1sc_Q_bkup,tmps)
      |       set_param(gcb,'fltCC1sc_Q',tmps);
      |     end
      |   end
      |   if isnan(fltCC2sc_Q)
      |     if ~strcmp(fltCC2sc_Q_bkup,'0')
      |       set_param(gcb,'fltCC2sc_Q','0');
      |     end
      |   else
      |     tmps=num2str(fltCC2sc_Q);
      |     if ~strcmp(fltCC2sc_Q_bkup,tmps)
      |       set_param(gcb,'fltCC2sc_Q',tmps);
      |     end
      |   end
      |   if isnan(fltUpperLimit_Q)
      |     if ~strcmp(fltUpperLimit_Q_bkup,'0')
      |       set_param(gcb,'fltUpperLimit_Q','0');
      |     end
      |   else
      |     tmps=num2str(fltUpperLimit_Q);
      |     if ~strcmp(fltUpperLimit_Q_bkup,tmps)
      |       set_param(gcb,'fltUpperLimit_Q',tmps);
      |     end
      |   end
      |   if isnan(fltLowerLimit_Q)
      |     if ~strcmp(fltLowerLimit_Q_bkup,'0')
      |       set_param(gcb,'fltLowerLimit_Q','0');
      |     end
      |   else
      |     tmps=num2str(fltLowerLimit_Q);
      |     if ~strcmp(fltLowerLimit_Q_bkup,tmps)
      |       set_param(gcb,'fltLowerLimit_Q',tmps);
      |     end
      |   end
      | end
      mask Callback polepairs:
      | autoCalcEn=get_param(gcb,'autoCalcEn');
      | if strcmp(autoCalcEn,'on')
      |   SampleTime=Simulink.data.evalinGlobal(bdroot,get_param(gcb,'SampleTime'));
      |   if (SampleTime==-1)
      |     SampleTime=str2double(get_param(gcb,'SampleTime_1'));
      |   end
      |   fltIGain_bkup=get_param(gcb,'fltIGain');
      |   fltUGain_bkup=get_param(gcb,'fltUGain');
      |   fltWIGain_bkup=get_param(gcb,'fltWIGain');
      |   fltEGain_bkup=get_param(gcb,'fltEGain');
      |   fltCC1sc_D_bkup=get_param(gcb,'fltCC1sc_D');
      |   fltCC2sc_D_bkup=get_param(gcb,'fltCC2sc_D');
      |   fltUpperLimit_D_bkup=get_param(gcb,'fltUpperLimit_D');
      |   fltLowerLimit_D_bkup=get_param(gcb,'fltLowerLimit_D');
      |   fltCC1sc_Q_bkup=get_param(gcb,'fltCC1sc_Q');
      |   fltCC2sc_Q_bkup=get_param(gcb,'fltCC2sc_Q');
      |   fltUpperLimit_Q_bkup=get_param(gcb,'fltUpperLimit_Q');
      |   fltLowerLimit_Q_bkup=get_param(gcb,'fltLowerLimit_Q');
      |   intmethod=get_param(gcb,'intmethod');
      |   if0=Simulink.data.evalinGlobal(bdroot,get_param(gcb,'if0'));
      |   iksi=Simulink.data.evalinGlobal(bdroot,get_param(gcb,'iksi'));
      |   Ld=Simulink.data.evalinGlobal(bdroot,get_param(gcb,'Ld'));
      |   Lq=Simulink.data.evalinGlobal(bdroot,get_param(gcb,'Lq'));
      |   Rs=Simulink.data.evalinGlobal(bdroot,get_param(gcb,'Rs'));
      |   mechspeed=Simulink.data.evalinGlobal(bdroot,get_param(gcb,'mechspeed'));
      |   polepairs=Simulink.data.evalinGlobal(bdroot,get_param(gcb,'polepairs'));
      |   if (if0<=0)
      |     warning('Natural frequency f0 must be positive.');
      |   end
      |   if (iksi<=0)
      |     warning('Current loop attenuation must be positive.');
      |   end
      |   if (iksi>1)
      |     warning('Current loop attenuation must not exceed 1.');
      |   end
      |   if (Ld<=0)
      |     warning('Inductance Ld must be positive.');
      |   end
      |   if (Lq<=0)
      |     warning('Inductance Lq must be positive.');
      |   end
      |   if (Rs<0)
      |     warning('Resistance Rs must be non-negative.');
      |   end
      |   if (mechspeed<=0)
      |     warning('Max. speed must be positive.');
      |   end
      |   if (polepairs<1)
      |     warning('Number of pole pairs must be a natural number (1, 2, 3, ...).');
      |   end
      |   if (round(polepairs)~=polepairs)
      |     warning('Number of pole pairs must be a natural number (1, 2, 3, ...).');
      |   end
      |   w0=6.283185307179586*if0;
      |   pgain=2.0*iksi*w0*Ld-Rs;
      |   igain=w0*w0*Ld;
      |   if strcmp(intmethod,'Forward Rectangular')
      |     cc1=pgain;
      |     cc2=-pgain+igain*SampleTime;
      |   else
      |     if strcmp(intmethod,'Backward Rectangular')
      |       cc1=pgain+igain*SampleTime;
      |       cc2=-pgain;
      |     else
      |       cc1=pgain+igain*SampleTime*0.5;
      |       cc2=-pgain+igain*SampleTime*0.5;
      |     end
      |   end
      |   fltCC1sc_D=cc1;
      |   fltCC2sc_D=cc2;
      |   fltCC1sc_Q=fltCC1sc_D;
      |   fltCC2sc_Q=fltCC2sc_D;
      |   fltLowerLimit_D=-1000000.0;
      |   fltUpperLimit_D=1000000.0;
      |   fltLowerLimit_Q=fltLowerLimit_D;
      |   fltUpperLimit_Q=fltUpperLimit_D;
      |   fltIGain=(2.0*Ld-SampleTime*Rs)/(2.0*Ld+SampleTime*Rs);
      |   fltUGain=SampleTime/(2.0*Ld+SampleTime*Rs);
      |   fltWIGain=SampleTime*Lq/(2.0*Ld+SampleTime*Rs);
      |   fltEGain=SampleTime/(2.0*Ld+SampleTime*Rs);
      |   if isnan(fltIGain)
      |     if ~strcmp(fltIGain_bkup,'0')
      |       set_param(gcb,'fltIGain','0');
      |     end
      |   else
      |     tmps=num2str(fltIGain);
      |     if ~strcmp(fltIGain_bkup,tmps)
      |       set_param(gcb,'fltIGain',tmps);
      |     end
      |   end
      |   if isnan(fltUGain)
      |     if ~strcmp(fltUGain_bkup,'0')
      |       set_param(gcb,'fltUGain','0');
      |     end
      |   else
      |     tmps=num2str(fltUGain);
      |     if ~strcmp(fltUGain_bkup,tmps)
      |       set_param(gcb,'fltUGain',tmps);
      |     end
      |   end
      |   if isnan(fltWIGain)
      |     if ~strcmp(fltWIGain_bkup,'0')
      |       set_param(gcb,'fltWIGain','0');
      |     end
      |   else
      |     tmps=num2str(fltWIGain);
      |     if ~strcmp(fltWIGain_bkup,tmps)
      |       set_param(gcb,'fltWIGain',tmps);
      |     end
      |   end
      |   if isnan(fltEGain)
      |     if ~strcmp(fltEGain_bkup,'0')
      |       set_param(gcb,'fltEGain','0');
      |     end
      |   else
      |     tmps=num2str(fltEGain);
      |     if ~strcmp(fltEGain_bkup,tmps)
      |       set_param(gcb,'fltEGain',tmps);
      |     end
      |   end
      |   if isnan(fltCC1sc_D)
      |     if ~strcmp(fltCC1sc_D_bkup,'0')
      |       set_param(gcb,'fltCC1sc_D','0');
      |     end
      |   else
      |     tmps=num2str(fltCC1sc_D);
      |     if ~strcmp(fltCC1sc_D_bkup,tmps)
      |       set_param(gcb,'fltCC1sc_D',tmps);
      |     end
      |   end
      |   if isnan(fltCC2sc_D)
      |     if ~strcmp(fltCC2sc_D_bkup,'0')
      |       set_param(gcb,'fltCC2sc_D','0');
      |     end
      |   else
      |     tmps=num2str(fltCC2sc_D);
      |     if ~strcmp(fltCC2sc_D_bkup,tmps)
      |       set_param(gcb,'fltCC2sc_D',tmps);
      |     end
      |   end
      |   if isnan(fltUpperLimit_D)
      |     if ~strcmp(fltUpperLimit_D_bkup,'0')
      |       set_param(gcb,'fltUpperLimit_D','0');
      |     end
      |   else
      |     tmps=num2str(fltUpperLimit_D);
      |     if ~strcmp(fltUpperLimit_D_bkup,tmps)
      |       set_param(gcb,'fltUpperLimit_D',tmps);
      |     end
      |   end
      |   if isnan(fltLowerLimit_D)
      |     if ~strcmp(fltLowerLimit_D_bkup,'0')
      |       set_param(gcb,'fltLowerLimit_D','0');
      |     end
      |   else
      |     tmps=num2str(fltLowerLimit_D);
      |     if ~strcmp(fltLowerLimit_D_bkup,tmps)
      |       set_param(gcb,'fltLowerLimit_D',tmps);
      |     end
      |   end
      |   if isnan(fltCC1sc_Q)
      |     if ~strcmp(fltCC1sc_Q_bkup,'0')
      |       set_param(gcb,'fltCC1sc_Q','0');
      |     end
      |   else
      |     tmps=num2str(fltCC1sc_Q);
      |     if ~strcmp(fltCC1sc_Q_bkup,tmps)
      |       set_param(gcb,'fltCC1sc_Q',tmps);
      |     end
      |   end
      |   if isnan(fltCC2sc_Q)
      |     if ~strcmp(fltCC2sc_Q_bkup,'0')
      |       set_param(gcb,'fltCC2sc_Q','0');
      |     end
      |   else
      |     tmps=num2str(fltCC2sc_Q);
      |     if ~strcmp(fltCC2sc_Q_bkup,tmps)
      |       set_param(gcb,'fltCC2sc_Q',tmps);
      |     end
      |   end
      |   if isnan(fltUpperLimit_Q)
      |     if ~strcmp(fltUpperLimit_Q_bkup,'0')
      |       set_param(gcb,'fltUpperLimit_Q','0');
      |     end
      |   else
      |     tmps=num2str(fltUpperLimit_Q);
      |     if ~strcmp(fltUpperLimit_Q_bkup,tmps)
      |       set_param(gcb,'fltUpperLimit_Q',tmps);
      |     end
      |   end
      |   if isnan(fltLowerLimit_Q)
      |     if ~strcmp(fltLowerLimit_Q_bkup,'0')
      |       set_param(gcb,'fltLowerLimit_Q','0');
      |     end
      |   else
      |     tmps=num2str(fltLowerLimit_Q);
      |     if ~strcmp(fltLowerLimit_Q_bkup,tmps)
      |       set_param(gcb,'fltLowerLimit_Q',tmps);
      |     end
      |   end
      | end
      mask Callback autoCalcEn:
      | maskStr=get_param(gcb,'showStates');
      | if strcmp(maskStr,'Hide (faster execution)')
      |   p=Simulink.Mask.get(gcb);
      |   autoCalcEn=get_param(gcb,'autoCalcEn');
      |   hintText=p.getDialogControl('timeHint');
      |   if strcmp(autoCalcEn,'on')
      |     param=p.getParameter('polepairs');
      |     if strcmp(param.Enabled,'off')
      |       SampleTime=Simulink.data.evalinGlobal(bdroot,get_param(gcb,'SampleTime'));
      |       if SampleTime==-1
      |         SampleTime=str2double(get_param(gcb,'SampleTime_1'));
      |         if isnan(SampleTime)
      |           hintText.Prompt=['Note: Implementation parameters cannot be calculated yet because the block''s inherited sample time is unknown. Simulink will update the sample time when you run the simulation.'];
      |         else
      |           hintText.Prompt=['Caution: Implementation parameters depend on inherited sample time. Make sure that the sample time of the block''s inputs corresponds to the sampling period in the target application.'];
      |         end
      |       else
      |         hintText.Prompt='Caution: Implementation parameters depend on the sample time. Make sure that the simulation time step corresponds to the sampling period in the target application.';
      |       end
      |       p=Simulink.Mask.get(gcb);
      |       param=p.getParameter('intmethod');
      |       param.set('Enabled','on');
      |       param=p.getParameter('if0');
      |       param.set('Enabled','on');
      |       param=p.getParameter('iksi');
      |       param.set('Enabled','on');
      |       param=p.getParameter('Ld');
      |       param.set('Enabled','on');
      |       param=p.getParameter('Lq');
      |       param.set('Enabled','on');
      |       param=p.getParameter('Rs');
      |       param.set('Enabled','on');
      |       param=p.getParameter('mechspeed');
      |       param.set('Enabled','on');
      |       param=p.getParameter('polepairs');
      |       param.set('Enabled','on');
      |     else
      |       SampleTime=Simulink.data.evalinGlobal(bdroot,get_param(gcb,'SampleTime'));
      |       if SampleTime==-1
      |         SampleTime=str2double(get_param(gcb,'SampleTime_1'));
      |       end
      |     end
      |     fltIGain_bkup=get_param(gcb,'fltIGain');
      |     fltUGain_bkup=get_param(gcb,'fltUGain');
      |     fltWIGain_bkup=get_param(gcb,'fltWIGain');
      |     fltEGain_bkup=get_param(gcb,'fltEGain');
      |     fltCC1sc_D_bkup=get_param(gcb,'fltCC1sc_D');
      |     fltCC2sc_D_bkup=get_param(gcb,'fltCC2sc_D');
      |     fltUpperLimit_D_bkup=get_param(gcb,'fltUpperLimit_D');
      |     fltLowerLimit_D_bkup=get_param(gcb,'fltLowerLimit_D');
      |     fltCC1sc_Q_bkup=get_param(gcb,'fltCC1sc_Q');
      |     fltCC2sc_Q_bkup=get_param(gcb,'fltCC2sc_Q');
      |     fltUpperLimit_Q_bkup=get_param(gcb,'fltUpperLimit_Q');
      |     fltLowerLimit_Q_bkup=get_param(gcb,'fltLowerLimit_Q');
      |     intmethod=get_param(gcb,'intmethod');
      |     if0=Simulink.data.evalinGlobal(bdroot,get_param(gcb,'if0'));
      |     iksi=Simulink.data.evalinGlobal(bdroot,get_param(gcb,'iksi'));
      |     Ld=Simulink.data.evalinGlobal(bdroot,get_param(gcb,'Ld'));
      |     Lq=Simulink.data.evalinGlobal(bdroot,get_param(gcb,'Lq'));
      |     Rs=Simulink.data.evalinGlobal(bdroot,get_param(gcb,'Rs'));
      |     mechspeed=Simulink.data.evalinGlobal(bdroot,get_param(gcb,'mechspeed'));
      |     polepairs=Simulink.data.evalinGlobal(bdroot,get_param(gcb,'polepairs'));
      |     if (if0<=0)
      |       warning('Natural frequency f0 must be positive.');
      |     end
      |     if (iksi<=0)
      |       warning('Current loop attenuation must be positive.');
      |     end
      |     if (iksi>1)
      |       warning('Current loop attenuation must not exceed 1.');
      |     end
      |     if (Ld<=0)
      |       warning('Inductance Ld must be positive.');
      |     end
      |     if (Lq<=0)
      |       warning('Inductance Lq must be positive.');
      |     end
      |     if (Rs<0)
      |       warning('Resistance Rs must be non-negative.');
      |     end
      |     if (mechspeed<=0)
      |       warning('Max. speed must be positive.');
      |     end
      |     if (polepairs<1)
      |       warning('Number of pole pairs must be a natural number (1, 2, 3, ...).');
      |     end
      |     if (round(polepairs)~=polepairs)
      |       warning('Number of pole pairs must be a natural number (1, 2, 3, ...).');
      |     end
      |     w0=6.283185307179586*if0;
      |     pgain=2.0*iksi*w0*Ld-Rs;
      |     igain=w0*w0*Ld;
      |     if strcmp(intmethod,'Forward Rectangular')
      |       cc1=pgain;
      |       cc2=-pgain+igain*SampleTime;
      |     else
      |       if strcmp(intmethod,'Backward Rectangular')
      |         cc1=pgain+igain*SampleTime;
      |         cc2=-pgain;
      |       else
      |         cc1=pgain+igain*SampleTime*0.5;
      |         cc2=-pgain+igain*SampleTime*0.5;
      |       end
      |     end
      |     fltCC1sc_D=cc1;
      |     fltCC2sc_D=cc2;
      |     fltCC1sc_Q=fltCC1sc_D;
      |     fltCC2sc_Q=fltCC2sc_D;
      |     fltLowerLimit_D=-1000000.0;
      |     fltUpperLimit_D=1000000.0;
      |     fltLowerLimit_Q=fltLowerLimit_D;
      |     fltUpperLimit_Q=fltUpperLimit_D;
      |     fltIGain=(2.0*Ld-SampleTime*Rs)/(2.0*Ld+SampleTime*Rs);
      |     fltUGain=SampleTime/(2.0*Ld+SampleTime*Rs);
      |     fltWIGain=SampleTime*Lq/(2.0*Ld+SampleTime*Rs);
      |     fltEGain=SampleTime/(2.0*Ld+SampleTime*Rs);
      |     if isnan(fltIGain)
      |       if ~strcmp(fltIGain_bkup,'0')
      |         set_param(gcb,'fltIGain','0');
      |       end
      |     else
      |       tmps=num2str(fltIGain);
      |       if ~strcmp(fltIGain_bkup,tmps)
      |         set_param(gcb,'fltIGain',tmps);
      |       end
      |     end
      |     if isnan(fltUGain)
      |       if ~strcmp(fltUGain_bkup,'0')
      |         set_param(gcb,'fltUGain','0');
      |       end
      |     else
      |       tmps=num2str(fltUGain);
      |       if ~strcmp(fltUGain_bkup,tmps)
      |         set_param(gcb,'fltUGain',tmps);
      |       end
      |     end
      |     if isnan(fltWIGain)
      |       if ~strcmp(fltWIGain_bkup,'0')
      |         set_param(gcb,'fltWIGain','0');
      |       end
      |     else
      |       tmps=num2str(fltWIGain);
      |       if ~strcmp(fltWIGain_bkup,tmps)
      |         set_param(gcb,'fltWIGain',tmps);
      |       end
      |     end
      |     if isnan(fltEGain)
      |       if ~strcmp(fltEGain_bkup,'0')
      |         set_param(gcb,'fltEGain','0');
      |       end
      |     else
      |       tmps=num2str(fltEGain);
      |       if ~strcmp(fltEGain_bkup,tmps)
      |         set_param(gcb,'fltEGain',tmps);
      |       end
      |     end
      |     if isnan(fltCC1sc_D)
      |       if ~strcmp(fltCC1sc_D_bkup,'0')
      |         set_param(gcb,'fltCC1sc_D','0');
      |       end
      |     else
      |       tmps=num2str(fltCC1sc_D);
      |       if ~strcmp(fltCC1sc_D_bkup,tmps)
      |         set_param(gcb,'fltCC1sc_D',tmps);
      |       end
      |     end
      |     if isnan(fltCC2sc_D)
      |       if ~strcmp(fltCC2sc_D_bkup,'0')
      |         set_param(gcb,'fltCC2sc_D','0');
      |       end
      |     else
      |       tmps=num2str(fltCC2sc_D);
      |       if ~strcmp(fltCC2sc_D_bkup,tmps)
      |         set_param(gcb,'fltCC2sc_D',tmps);
      |       end
      |     end
      |     if isnan(fltUpperLimit_D)
      |       if ~strcmp(fltUpperLimit_D_bkup,'0')
      |         set_param(gcb,'fltUpperLimit_D','0');
      |       end
      |     else
      |       tmps=num2str(fltUpperLimit_D);
      |       if ~strcmp(fltUpperLimit_D_bkup,tmps)
      |         set_param(gcb,'fltUpperLimit_D',tmps);
      |       end
      |     end
      |     if isnan(fltLowerLimit_D)
      |       if ~strcmp(fltLowerLimit_D_bkup,'0')
      |         set_param(gcb,'fltLowerLimit_D','0');
      |       end
      |     else
      |       tmps=num2str(fltLowerLimit_D);
      |       if ~strcmp(fltLowerLimit_D_bkup,tmps)
      |         set_param(gcb,'fltLowerLimit_D',tmps);
      |       end
      |     end
      |     if isnan(fltCC1sc_Q)
      |       if ~strcmp(fltCC1sc_Q_bkup,'0')
      |         set_param(gcb,'fltCC1sc_Q','0');
      |       end
      |     else
      |       tmps=num2str(fltCC1sc_Q);
      |       if ~strcmp(fltCC1sc_Q_bkup,tmps)
      |         set_param(gcb,'fltCC1sc_Q',tmps);
      |       end
      |     end
      |     if isnan(fltCC2sc_Q)
      |       if ~strcmp(fltCC2sc_Q_bkup,'0')
      |         set_param(gcb,'fltCC2sc_Q','0');
      |       end
      |     else
      |       tmps=num2str(fltCC2sc_Q);
      |       if ~strcmp(fltCC2sc_Q_bkup,tmps)
      |         set_param(gcb,'fltCC2sc_Q',tmps);
      |       end
      |     end
      |     if isnan(fltUpperLimit_Q)
      |       if ~strcmp(fltUpperLimit_Q_bkup,'0')
      |         set_param(gcb,'fltUpperLimit_Q','0');
      |       end
      |     else
      |       tmps=num2str(fltUpperLimit_Q);
      |       if ~strcmp(fltUpperLimit_Q_bkup,tmps)
      |         set_param(gcb,'fltUpperLimit_Q',tmps);
      |       end
      |     end
      |     if isnan(fltLowerLimit_Q)
      |       if ~strcmp(fltLowerLimit_Q_bkup,'0')
      |         set_param(gcb,'fltLowerLimit_Q','0');
      |       end
      |     else
      |       tmps=num2str(fltLowerLimit_Q);
      |       if ~strcmp(fltLowerLimit_Q_bkup,tmps)
      |         set_param(gcb,'fltLowerLimit_Q',tmps);
      |       end
      |     end
      |   else
      |     param=p.getParameter('polepairs');
      |     if strcmp(param.Enabled,'on')
      |       hintText.Prompt='Caution: Implementation parameters are fixed.';
      |       p=Simulink.Mask.get(gcb);
      |       param=p.getParameter('intmethod');
      |       param.set('Enabled','off');
      |       param=p.getParameter('if0');
      |       param.set('Enabled','off');
      |       param=p.getParameter('iksi');
      |       param.set('Enabled','off');
      |       param=p.getParameter('Ld');
      |       param.set('Enabled','off');
      |       param=p.getParameter('Lq');
      |       param.set('Enabled','off');
      |       param=p.getParameter('Rs');
      |       param.set('Enabled','off');
      |       param=p.getParameter('mechspeed');
      |       param.set('Enabled','off');
      |       param=p.getParameter('polepairs');
      |       param.set('Enabled','off');
      |     end
      |   end
      | end
      mask DialogControl CompBut Prompt: Recalculate sample times
      mask DialogControl CompBut Tooltip: Simulink updates the sample times of all blocks when the simulation is run. This button will update the sample times now.
      mask DialogControl CompBut Callback:
      | btn=questdlg('This will apply all changes in all open dialog boxes and update the schematic. Do you want to proceed?','Apply all changes','Continue','Cancel','Continue');
      | if strcmp(btn,'Continue')
      |   dlgs=DAStudio.ToolRoot.getOpenDialogs;
      |   for i=1:length(dlgs)
      |     dlgs(i).apply;
      |   end
      |   try
      |     SampleTime_1=str2double(get_param(gcb,'SampleTime_1'));
      |     ts=Simulink.Block.getSampleTimes(gcb);
      |     ts=ts(1).Value(1);
      |     if (SampleTime_1 ~= ts)
      |       SampleTime_1=ts;
      |       set_param(gcb,'SampleTime_1',num2str(ts));
      |       autoCalcEn=get_param(gcb,'autoCalcEn');
      |       if strcmp(autoCalcEn,'on')
      |         SampleTime=Simulink.data.evalinGlobal(bdroot,get_param(gcb,'SampleTime'));
      |         p=Simulink.Mask.get(gcb);
      |         hintText=p.getDialogControl('timeHint');
      |         if SampleTime==-1
      |           SampleTime=SampleTime_1;
      |           hintText.Prompt='Caution: Implementation parameters depend on inherited sample time. Make sure that the sample time of the block''s inputs corresponds to the sampling period in the target application.';
      |         else
      |           hintText.Prompt='Caution: Implementation parameters depend on the sample time. Make sure that the simulation time step corresponds to the sampling period in the target application.';
      |         end
      |         fltIGain_bkup=get_param(gcb,'fltIGain');
      |         fltUGain_bkup=get_param(gcb,'fltUGain');
      |         fltWIGain_bkup=get_param(gcb,'fltWIGain');
      |         fltEGain_bkup=get_param(gcb,'fltEGain');
      |         fltCC1sc_D_bkup=get_param(gcb,'fltCC1sc_D');
      |         fltCC2sc_D_bkup=get_param(gcb,'fltCC2sc_D');
      |         fltUpperLimit_D_bkup=get_param(gcb,'fltUpperLimit_D');
      |         fltLowerLimit_D_bkup=get_param(gcb,'fltLowerLimit_D');
      |         fltCC1sc_Q_bkup=get_param(gcb,'fltCC1sc_Q');
      |         fltCC2sc_Q_bkup=get_param(gcb,'fltCC2sc_Q');
      |         fltUpperLimit_Q_bkup=get_param(gcb,'fltUpperLimit_Q');
      |         fltLowerLimit_Q_bkup=get_param(gcb,'fltLowerLimit_Q');
      |         intmethod=get_param(gcb,'intmethod');
      |         if0=Simulink.data.evalinGlobal(bdroot,get_param(gcb,'if0'));
      |         iksi=Simulink.data.evalinGlobal(bdroot,get_param(gcb,'iksi'));
      |         Ld=Simulink.data.evalinGlobal(bdroot,get_param(gcb,'Ld'));
      |         Lq=Simulink.data.evalinGlobal(bdroot,get_param(gcb,'Lq'));
      |         Rs=Simulink.data.evalinGlobal(bdroot,get_param(gcb,'Rs'));
      |         mechspeed=Simulink.data.evalinGlobal(bdroot,get_param(gcb,'mechspeed'));
      |         polepairs=Simulink.data.evalinGlobal(bdroot,get_param(gcb,'polepairs'));
      |         if (if0<=0)
      |           warning('Natural frequency f0 must be positive.');
      |         end
      |         if (iksi<=0)
      |           warning('Current loop attenuation must be positive.');
      |         end
      |         if (iksi>1)
      |           warning('Current loop attenuation must not exceed 1.');
      |         end
      |         if (Ld<=0)
      |           warning('Inductance Ld must be positive.');
      |         end
      |         if (Lq<=0)
      |           warning('Inductance Lq must be positive.');
      |         end
      |         if (Rs<0)
      |           warning('Resistance Rs must be non-negative.');
      |         end
      |         if (mechspeed<=0)
      |           warning('Max. speed must be positive.');
      |         end
      |         if (polepairs<1)
      |           warning('Number of pole pairs must be a natural number (1, 2, 3, ...).');
      |         end
      |         if (round(polepairs)~=polepairs)
      |           warning('Number of pole pairs must be a natural number (1, 2, 3, ...).');
      |         end
      |         w0=6.283185307179586*if0;
      |         pgain=2.0*iksi*w0*Ld-Rs;
      |         igain=w0*w0*Ld;
      |         if strcmp(intmethod,'Forward Rectangular')
      |           cc1=pgain;
      |           cc2=-pgain+igain*SampleTime;
      |         else
      |           if strcmp(intmethod,'Backward Rectangular')
      |             cc1=pgain+igain*SampleTime;
      |             cc2=-pgain;
      |           else
      |             cc1=pgain+igain*SampleTime*0.5;
      |             cc2=-pgain+igain*SampleTime*0.5;
      |           end
      |         end
      |         fltCC1sc_D=cc1;
      |         fltCC2sc_D=cc2;
      |         fltCC1sc_Q=fltCC1sc_D;
      |         fltCC2sc_Q=fltCC2sc_D;
      |         fltLowerLimit_D=-1000000.0;
      |         fltUpperLimit_D=1000000.0;
      |         fltLowerLimit_Q=fltLowerLimit_D;
      |         fltUpperLimit_Q=fltUpperLimit_D;
      |         fltIGain=(2.0*Ld-SampleTime*Rs)/(2.0*Ld+SampleTime*Rs);
      |         fltUGain=SampleTime/(2.0*Ld+SampleTime*Rs);
      |         fltWIGain=SampleTime*Lq/(2.0*Ld+SampleTime*Rs);
      |         fltEGain=SampleTime/(2.0*Ld+SampleTime*Rs);
      |         if isnan(fltIGain)
      |           if ~strcmp(fltIGain_bkup,'0')
      |             set_param(gcb,'fltIGain','0');
      |           end
      |         else
      |           tmps=num2str(fltIGain);
      |           if ~strcmp(fltIGain_bkup,tmps)
      |             set_param(gcb,'fltIGain',tmps);
      |           end
      |         end
      |         if isnan(fltUGain)
      |           if ~strcmp(fltUGain_bkup,'0')
      |             set_param(gcb,'fltUGain','0');
      |           end
      |         else
      |           tmps=num2str(fltUGain);
      |           if ~strcmp(fltUGain_bkup,tmps)
      |             set_param(gcb,'fltUGain',tmps);
      |           end
      |         end
      |         if isnan(fltWIGain)
      |           if ~strcmp(fltWIGain_bkup,'0')
      |             set_param(gcb,'fltWIGain','0');
      |           end
      |         else
      |           tmps=num2str(fltWIGain);
      |           if ~strcmp(fltWIGain_bkup,tmps)
      |             set_param(gcb,'fltWIGain',tmps);
      |           end
      |         end
      |         if isnan(fltEGain)
      |           if ~strcmp(fltEGain_bkup,'0')
      |             set_param(gcb,'fltEGain','0');
      |           end
      |         else
      |           tmps=num2str(fltEGain);
      |           if ~strcmp(fltEGain_bkup,tmps)
      |             set_param(gcb,'fltEGain',tmps);
      |           end
      |         end
      |         if isnan(fltCC1sc_D)
      |           if ~strcmp(fltCC1sc_D_bkup,'0')
      |             set_param(gcb,'fltCC1sc_D','0');
      |           end
      |         else
      |           tmps=num2str(fltCC1sc_D);
      |           if ~strcmp(fltCC1sc_D_bkup,tmps)
      |             set_param(gcb,'fltCC1sc_D',tmps);
      |           end
      |         end
      |         if isnan(fltCC2sc_D)
      |           if ~strcmp(fltCC2sc_D_bkup,'0')
      |             set_param(gcb,'fltCC2sc_D','0');
      |           end
      |         else
      |           tmps=num2str(fltCC2sc_D);
      |           if ~strcmp(fltCC2sc_D_bkup,tmps)
      |             set_param(gcb,'fltCC2sc_D',tmps);
      |           end
      |         end
      |         if isnan(fltUpperLimit_D)
      |           if ~strcmp(fltUpperLimit_D_bkup,'0')
      |             set_param(gcb,'fltUpperLimit_D','0');
      |           end
      |         else
      |           tmps=num2str(fltUpperLimit_D);
      |           if ~strcmp(fltUpperLimit_D_bkup,tmps)
      |             set_param(gcb,'fltUpperLimit_D',tmps);
      |           end
      |         end
      |         if isnan(fltLowerLimit_D)
      |           if ~strcmp(fltLowerLimit_D_bkup,'0')
      |             set_param(gcb,'fltLowerLimit_D','0');
      |           end
      |         else
      |           tmps=num2str(fltLowerLimit_D);
      |           if ~strcmp(fltLowerLimit_D_bkup,tmps)
      |             set_param(gcb,'fltLowerLimit_D',tmps);
      |           end
      |         end
      |         if isnan(fltCC1sc_Q)
      |           if ~strcmp(fltCC1sc_Q_bkup,'0')
      |             set_param(gcb,'fltCC1sc_Q','0');
      |           end
      |         else
      |           tmps=num2str(fltCC1sc_Q);
      |           if ~strcmp(fltCC1sc_Q_bkup,tmps)
      |             set_param(gcb,'fltCC1sc_Q',tmps);
      |           end
      |         end
      |         if isnan(fltCC2sc_Q)
      |           if ~strcmp(fltCC2sc_Q_bkup,'0')
      |             set_param(gcb,'fltCC2sc_Q','0');
      |           end
      |         else
      |           tmps=num2str(fltCC2sc_Q);
      |           if ~strcmp(fltCC2sc_Q_bkup,tmps)
      |             set_param(gcb,'fltCC2sc_Q',tmps);
      |           end
      |         end
      |         if isnan(fltUpperLimit_Q)
      |           if ~strcmp(fltUpperLimit_Q_bkup,'0')
      |             set_param(gcb,'fltUpperLimit_Q','0');
      |           end
      |         else
      |           tmps=num2str(fltUpperLimit_Q);
      |           if ~strcmp(fltUpperLimit_Q_bkup,tmps)
      |             set_param(gcb,'fltUpperLimit_Q',tmps);
      |           end
      |         end
      |         if isnan(fltLowerLimit_Q)
      |           if ~strcmp(fltLowerLimit_Q_bkup,'0')
      |             set_param(gcb,'fltLowerLimit_Q','0');
      |           end
      |         else
      |           tmps=num2str(fltLowerLimit_Q);
      |           if ~strcmp(fltLowerLimit_Q_bkup,tmps)
      |             set_param(gcb,'fltLowerLimit_Q',tmps);
      |           end
      |         end
      |       end
      |     end
      |   catch
      |    warning(['Sample time cannot be calculated for the block ' gcb])
      |   end
      | end
      mask DialogControl timeHint Prompt: Note: Implementation parameters cannot be calculated yet because the block's inherited sample time is unknown. Simulink will update the sample time when you run the simulation.
      mask Display:
      | color('black');
      | pos = get_param(gcb, 'Position');
      | width = pos(3) - pos(1);
      | height = pos(4) - pos(2);
      | tX=width/2;
      | tY=height - 25;
      | color('black');
      | text(tX,tY, 'AMCLIB_BemfObsrvDQ_FLT', 'horizontalAlignment', 'center');
      | if showStates == 2
      |   color('red');
      |   text(tX,tY - 20, ['debugging mode' char(13) char(10) '(limited performance)'], 'horizontalAlignment', 'center');
      | end
  AMCLIB_CurrentLoopPIp_FLT : Subsystem  StartFcn=|  TreatAsAtomicUnit=on  mask(AMCLIB_CurrentLoopPIp_FLT){showStates=Hide (faster execution), resetStatesEnable=Pre-set according to the first set of inputs after reset, SampleTime=-1, if0=350, iksi=1, Ld=3e-4, Lq=3e-4, Rs=0.33, autoCalcEn=on, fltPropGain_D=0, fltIntegGain_D=0, fltPropGain_Q=0, fltIntegGain_Q=0, SampleTime_1=NaN}
      | ts=get_param(gcb,'CompiledSampleTime');
      | if iscell(ts)
      |   ts=ts{1};
      |   if iscell(ts)
      |     ts=ts{1};
      |   end
      | end
      | ts=ts(1);
      | set_param(gcb,'SampleTime_1',num2str(ts));
      | p=Simulink.Mask.get(gcb);
      | hintText=p.getDialogControl('timeHint');
      | SampleTime=Simulink.data.evalinGlobal(bdroot,get_param(gcb,'SampleTime'));
      | p=Simulink.Mask.get(gcb);
      | autoCalcEn=get_param(gcb,'autoCalcEn');
      | if strcmp(autoCalcEn,'on')
      |   if SampleTime==-1
      |     hintText.Prompt='Caution: Implementation parameters depend on inherited sample time. Make sure that the sample time of the block''s inputs corresponds to the sampling period in the target application.';
      |   else
      |     hintText.Prompt='Caution: Implementation parameters depend on the sample time. Make sure that the simulation time step corresponds to the sampling period in the target application.';
      |   end
      |   SampleTime=ts;
      |   fltPropGain_D_bkup=get_param(gcb,'fltPropGain_D');
      |   fltIntegGain_D_bkup=get_param(gcb,'fltIntegGain_D');
      |   fltPropGain_Q_bkup=get_param(gcb,'fltPropGain_Q');
      |   fltIntegGain_Q_bkup=get_param(gcb,'fltIntegGain_Q');
      |   if0=Simulink.data.evalinGlobal(bdroot,get_param(gcb,'if0'));
      |   iksi=Simulink.data.evalinGlobal(bdroot,get_param(gcb,'iksi'));
      |   Ld=Simulink.data.evalinGlobal(bdroot,get_param(gcb,'Ld'));
      |   Lq=Simulink.data.evalinGlobal(bdroot,get_param(gcb,'Lq'));
      |   Rs=Simulink.data.evalinGlobal(bdroot,get_param(gcb,'Rs'));
      |   if (if0<=0)
      |     warning('Natural frequency f0 must be positive.');
      |   end
      |   if (iksi<=0)
      |     warning('Current loop attenuation must be positive.');
      |   end
      |   if (iksi>1)
      |     warning('Current loop attenuation must not exceed 1.');
      |   end
      |   if (Ld<=0)
      |     warning('Inductance Ld must be positive.');
      |   end
      |   if (Lq<=0)
      |     warning('Inductance Lq must be positive.');
      |   end
      |   if (Rs<0)
      |     warning('Resistance Rs must be non-negative.');
      |   end
      |   w0=6.283185307179586*if0;
      |   pgainD=2.0*iksi*w0*Ld-Rs;
      |   igainD=w0*w0*Ld;
      |   pgainQ=2.0*iksi*w0*Lq-Rs;
      |   igainQ=w0*w0*Lq;
      |   fltPropGain_D=pgainD;
      |   fltIntegGain_D=igainD*SampleTime*0.5;
      |   fltPropGain_Q=pgainQ;
      |   fltIntegGain_Q=igainQ*SampleTime*0.5;
      |   if isnan(fltPropGain_D)
      |     if ~strcmp(fltPropGain_D_bkup,'0')
      |       set_param(gcb,'fltPropGain_D','0');
      |     end
      |   else
      |     tmps=num2str(fltPropGain_D);
      |     if ~strcmp(fltPropGain_D_bkup,tmps)
      |       set_param(gcb,'fltPropGain_D',tmps);
      |     end
      |   end
      |   if isnan(fltIntegGain_D)
      |     if ~strcmp(fltIntegGain_D_bkup,'0')
      |       set_param(gcb,'fltIntegGain_D','0');
      |     end
      |   else
      |     tmps=num2str(fltIntegGain_D);
      |     if ~strcmp(fltIntegGain_D_bkup,tmps)
      |       set_param(gcb,'fltIntegGain_D',tmps);
      |     end
      |   end
      |   if isnan(fltPropGain_Q)
      |     if ~strcmp(fltPropGain_Q_bkup,'0')
      |       set_param(gcb,'fltPropGain_Q','0');
      |     end
      |   else
      |     tmps=num2str(fltPropGain_Q);
      |     if ~strcmp(fltPropGain_Q_bkup,tmps)
      |       set_param(gcb,'fltPropGain_Q',tmps);
      |     end
      |   end
      |   if isnan(fltIntegGain_Q)
      |     if ~strcmp(fltIntegGain_Q_bkup,'0')
      |       set_param(gcb,'fltIntegGain_Q','0');
      |     end
      |   else
      |     tmps=num2str(fltIntegGain_Q);
      |     if ~strcmp(fltIntegGain_Q_bkup,tmps)
      |       set_param(gcb,'fltIntegGain_Q',tmps);
      |     end
      |   end
      | end
      mask prompts: showStates "Show internal states:"; resetStatesEnable "Internal state after reset"; SampleTime "Sample time (-1 for inherited):"; if0 "Current loop natural frequency f0 [Hz]:"; iksi "Current loop attenuation ξ:"; Ld "D-axis stator inductance Ld [H]"; Lq "Q-axis stator inductance Lq [H]"; Rs "Winding resistance Rs [ohm]:"; autoCalcEn "Calculate implementation parameters from physical parameters"; fltPropGain_D "Proportional gain of the D-axis PI controller"; fltIntegGain_D "Integral gain of the D-axis PI controller"; fltPropGain_Q "Proportional gain of the Q-axis PI controller"; fltIntegGain_Q "Integral gain of the Q-axis PI controller"; SampleTime_1 "Discrete sample time:"
      mask help: Current control loop of the PMSM field-oriented control algorithm in single precision floating-point implementation. The current control loop contains two PI controllers in parallel form. This block supports re-initialization of the internal state during simulation. If the block is reset, the outputs of the PI controllers will be aligned with the inputs fltControllerPIpAWDOut_preset and fltControllerPIpAWQOut_preset. Refer to the AMMCLIB User's Guide for further details.
      mask init:
      | ddName = get_param(bdroot,'DataDictionary');
      | if length(ddName)==0
      |   set_param(bdroot,'DataDictionary','ammclib_types.sldd');
      | else
      |   dd = Simulink.data.dictionary.open(ddName);
      |   data = getSection(dd,'Design Data');
      |   if ~exist(data,'SWLIBS_2Syst_F16')
      |     addDataSource(dd,'ammclib_types.sldd');
      |     saveChanges(dd);
      |   end
      | end
      | 
      | if showStates == 1
      |   % hidden state variables
      |   if strcmp(get_param([gcb '/fltPropGain_D'], 'BlockType'), 'Inport')
      |     posblk = get_param(gcb, 'Position');
      | 
      |     pos = get_param([gcb, '/fltPropGain_D'], 'Position');
      |     orient = get_param([gcb, '/fltPropGain_D'], 'Orientation');
      |     delete_block([gcb, '/fltPropGain_D']);
      |     add_block('built-in/Ground', [gcb, '/fltPropGain_D'], 'Position', pos, 'Orientation', orient);
      | 
      |     pos = get_param([gcb, '/fltIntegGain_D'], 'Position');
      |     orient = get_param([gcb, '/fltIntegGain_D'], 'Orientation');
      |     delete_block([gcb, '/fltIntegGain_D']);
      |     add_block('built-in/Ground', [gcb, '/fltIntegGain_D'], 'Position', pos, 'Orientation', orient);
      | 
      |     pos = get_param([gcb, '/fltIntegPartK_1_D'], 'Position');
      |     orient = get_param([gcb, '/fltIntegPartK_1_D'], 'Orientation');
      |     delete_block([gcb, '/fltIntegPartK_1_D']);
      |     add_block('built-in/Ground', [gcb, '/fltIntegPartK_1_D'], 'Position', pos, 'Orientation', orient);
      | 
      |     pos = get_param([gcb, '/fltInK_1_D'], 'Position');
      |     orient = get_param([gcb, '/fltInK_1_D'], 'Orientation');
      |     delete_block([gcb, '/fltInK_1_D']);
      |     add_block('built-in/Ground', [gcb, '/fltInK_1_D'], 'Position', pos, 'Orientation', orient);
      | 
      |     pos = get_param([gcb, '/fltPropGain_Q'], 'Position');
      |     orient = get_param([gcb, '/fltPropGain_Q'], 'Orientation');
      |     delete_block([gcb, '/fltPropGain_Q']);
      |     add_block('built-in/Ground', [gcb, '/fltPropGain_Q'], 'Position', pos, 'Orientation', orient);
      | 
      |     pos = get_param([gcb, '/fltIntegGain_Q'], 'Position');
      |     orient = get_param([gcb, '/fltIntegGain_Q'], 'Orientation');
      |     delete_block([gcb, '/fltIntegGain_Q']);
      |     add_block('built-in/Ground', [gcb, '/fltIntegGain_Q'], 'Position', pos, 'Orientation', orient);
      | 
      |     pos = get_param([gcb, '/fltIntegPartK_1_Q'], 'Position');
      |     orient = get_param([gcb, '/fltIntegPartK_1_Q'], 'Orientation');
      |     delete_block([gcb, '/fltIntegPartK_1_Q']);
      |     add_block('built-in/Ground', [gcb, '/fltIntegPartK_1_Q'], 'Position', pos, 'Orientation', orient);
      | 
      |     pos = get_param([gcb, '/fltInK_1_Q'], 'Position');
      |     orient = get_param([gcb, '/fltInK_1_Q'], 'Orientation');
      |     delete_block([gcb, '/fltInK_1_Q']);
      |     add_block('built-in/Ground', [gcb, '/fltInK_1_Q'], 'Position', pos, 'Orientation', orient);
      | 
      | 
      |     pmask=Simulink.Mask.get(gcb);
      |     pctrl=pmask.getParameter('SampleTime');
      |     pctrl.set('TypeOptions',{'fltUDcBus/SampleTime','pIDQReq/SampleTime','pIDQFbck/SampleTime','fltControllerPIpAWDOut_preset/SampleTime','fltControllerPIpAWQOut_preset/SampleTime'});
      | 
      |     pos = get_param([gcb '/fltIntegPartK_1_D_Out'], 'Position');
      |     orient = get_param([gcb '/fltIntegPartK_1_D_Out'], 'Orientation');
      |     delete_block([gcb '/fltIntegPartK_1_D_Out']);
      |     add_block('built-in/Terminator', [gcb '/fltIntegPartK_1_D_Out'], 'Position', pos, 'Orientation', orient);
      | 
      |     pos = get_param([gcb '/fltInK_1_D_Out'], 'Position');
      |     orient = get_param([gcb '/fltInK_1_D_Out'], 'Orientation');
      |     delete_block([gcb '/fltInK_1_D_Out']);
      |     add_block('built-in/Terminator', [gcb '/fltInK_1_D_Out'], 'Position', pos, 'Orientation', orient);
      | 
      |     pos = get_param([gcb '/fltIntegPartK_1_Q_Out'], 'Position');
      |     orient = get_param([gcb '/fltIntegPartK_1_Q_Out'], 'Orientation');
      |     delete_block([gcb '/fltIntegPartK_1_Q_Out']);
      |     add_block('built-in/Terminator', [gcb '/fltIntegPartK_1_Q_Out'], 'Position', pos, 'Orientation', orient);
      | 
      |     pos = get_param([gcb '/fltInK_1_Q_Out'], 'Position');
      |     orient = get_param([gcb '/fltInK_1_Q_Out'], 'Orientation');
      |     delete_block([gcb '/fltInK_1_Q_Out']);
      |     add_block('built-in/Terminator', [gcb '/fltInK_1_Q_Out'], 'Position', pos, 'Orientation', orient);
      | 
      |     set_param([gcb '/fltUDcBus'], 'Port', '1');
      |     set_param([gcb '/pIDQReq'], 'Port', '2');
      |     set_param([gcb '/pIDQFbck'], 'Port', '3');
      |     set_param([gcb '/fltControllerPIpAWDOut_preset'], 'Port', '4');
      |     set_param([gcb '/fltControllerPIpAWQOut_preset'], 'Port', '5');
      | 
      |     tmpOutCnt=0;
      |     tmpOutCnt=tmpOutCnt+1;
      |     set_param([gcb '/pUDQReq'], 'Port', num2str(tmpOutCnt));
      |     tmpOutCnt=tmpOutCnt+1;
      |     set_param([gcb '/fltUQLim'], 'Port', num2str(tmpOutCnt));
      | 
      |     autoCalcEn=get_param(gcb,'autoCalcEn');
      |     if strcmp(autoCalcEn,'on')
      |       set_param(gcb,'MaskEnables',{'on','on','on','on','on','on','on','on','on','on','on','on','on','off'});
      |     else
      |       set_param(gcb,'MaskEnables',{'on','on','on','off','off','off','off','off','on','on','on','on','on','off'});
      |     end
      | 
      |     if (posblk(4) - posblk(2)) > 150
      |       height = 150;
      |       set_param(gcb,'Position',[posblk(1), posblk(2), posblk(3), posblk(2)+height])
      |     end
      |   end
      | else
      |   % shown state variables
      |   if strcmp(get_param([gcb '/fltPropGain_D'], 'BlockType'), 'Ground')
      |     posblk = get_param(gcb, 'Position');
      | 
      |     pos = get_param([gcb, '/fltPropGain_D'], 'Position');
      |     orient = get_param([gcb, '/fltPropGain_D'], 'Orientation');
      |     delete_block([gcb, '/fltPropGain_D']);
      |     add_block('built-in/Inport', [gcb, '/fltPropGain_D'], 'Position', pos, 'Orientation', orient, 'OutDataTypeStr', 'single');
      | 
      |     pos = get_param([gcb, '/fltIntegGain_D'], 'Position');
      |     orient = get_param([gcb, '/fltIntegGain_D'], 'Orientation');
      |     delete_block([gcb, '/fltIntegGain_D']);
      |     add_block('built-in/Inport', [gcb, '/fltIntegGain_D'], 'Position', pos, 'Orientation', orient, 'OutDataTypeStr', 'single');
      | 
      |     pos = get_param([gcb, '/fltIntegPartK_1_D'], 'Position');
      |     orient = get_param([gcb, '/fltIntegPartK_1_D'], 'Orientation');
      |     delete_block([gcb, '/fltIntegPartK_1_D']);
      |     add_block('built-in/Inport', [gcb, '/fltIntegPartK_1_D'], 'Position', pos, 'Orientation', orient, 'OutDataTypeStr', 'single');
      | 
      |     pos = get_param([gcb, '/fltInK_1_D'], 'Position');
      |     orient = get_param([gcb, '/fltInK_1_D'], 'Orientation');
